simulink model "35-Bus_Network_Electricity_Transmission_Model"  (R2023b)
settings: Solver=VariableStepAuto  StartTime=0.0  StopTime=10  RelTol=1e-3
undefined symbols (not defined in the file): D1, D11, Delta
libraries: spsSeriesRLCBranchLib x47, spsLoadFlowBusLib x35, spsThreePhaseSeriesRLCLoadLib x27, spsDistributedParametersLineLib x22, spsGenericPowerSystemStabilizerLib x20, spsThreePhaseTransformerTwoWindingsLib x19, spsThreePhaseVIMeasurementLib x13, spsSynchronousMachinepuStandardLib x10, spsExcitationSystemLib x10, spsHydraulicTurbineandGovernorLib x10, spsThreePhaseParallelRLCLoadLib x4, spsGroundLib x3
(part 5 of 7)

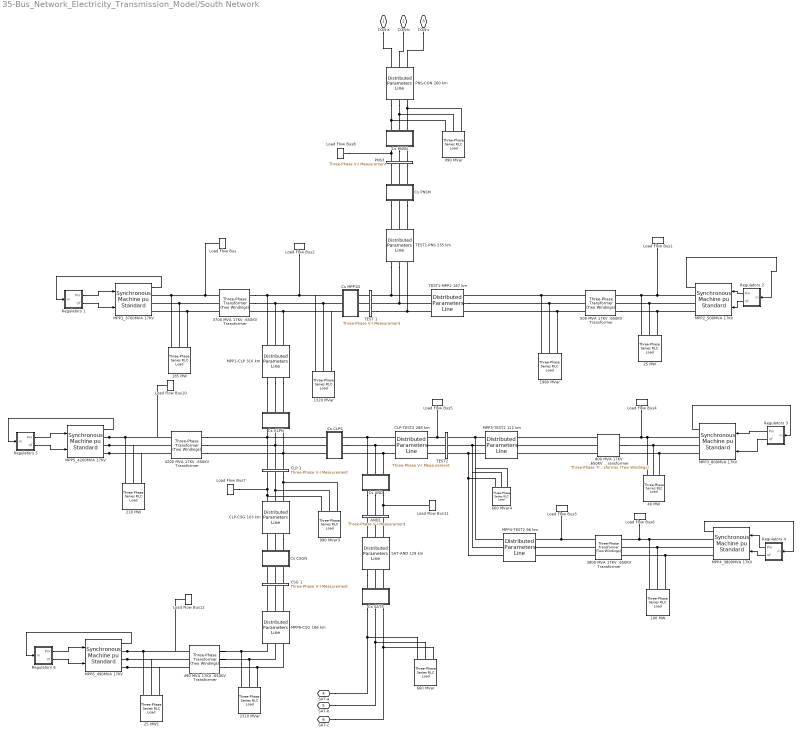
== system 35-Bus_Network_Electricity_Transmission_Model/South Network ==
  " SAT-AND 129 km" : spsDistributedParametersLineLib/Distributed Parameters Line  Phases=3  Length=129  Frequency=60  Resistance=[0.01273 0.3864]/6  Inductance="[0.9337e-3  4.1264e-3]/6"  Capacitance=[12.74e-9 7.751e-9]*6  x1=[-0.00078 -3.83682722016128e-12 0.674511153374435 -1.04249596847644;-0.00072 -3.77067090918174e-12 0.70818806056143 -1.04121442899321;-0.00066 -3.70258545329108e-12 0.741502645650831 -1.03940018496868;-0.0006 -3.63260568626661e-12 0.774437864285324 -1.03705416460361;-0.00054 -3.5607674110502e-12 0.806976866198483 -1.03417756816538;-0.00048 -3.48710738143088e-12 0.839103003835676 -1.03077186737387;-0.00042 -3.41166328324089e-12 0.870799840871265 -1.02683880464853;-0.00036 -3.3344737150749e-12 0.902051160617734 -1.02238039221694;-0.0003 -3.25557816854229e-12 0.932840974322442 -1.01739891108527;-0.00024 -3.17501700806249e-12 0.963153529347768 -1.01189690987132;-0.00018 -3.09283145021379e-12 0.992973317230448 -1.00587720350057;-0.00012 -3.00906354264621e-12 1.022285081616 -0.999342871766043;-6e-05 -2.9237561425691e-12 1.05107382606413 -0.992297257752584]  x2=[-0.00078 2.44939148388225e-11 -0.211095894428946 0.447209046200146;-0.00072 2.42785115163366e-11 -0.22627061958859 0.447871126318045;-0.00066 2.40506868587436e-11 -0.241329580518252 0.448304067292014;-0.0006 2.38105574253482e-11 -0.256265072775263 0.448507647621449;-0.00054 2.35582460708054e-11 -0.271069455085808 0.448481763150892;-0.00048 2.32938818822664e-11 -0.285735153254343 0.448226427123317;-0.00042 2.3017600113335e-11 -0.300254664038695 0.447741770173354;-0.00036 2.27295421148693e-11 -0.314620558988856 0.447028040260454;-0.0003 2.2429855262664e-11 -0.328825488247519 0.446085602542028;-0.00024 2.21186928820502e-11 -0.342862184310398 0.444914939186627;-0.00018 2.17962141694515e-11 -0.35672346574442 0.443516649127255;-0.00012 2.1462584110936e-11 -0.370402240861875 0.441891447754944;-6e-05 2.11179733978064e-11 -0.383891511348658 0.440040166552747]  x3=[-0.00078 4.92364553079132e-13 0.294721852728447 -0.0146104918256409;-0.00072 5.08483648349703e-13 0.292540672457794 -0.0101755439802829;-0.00066 5.24342593990081e-13 0.290209822973581 -0.00573539013860211;-0.0006 5.39933276270636e-13 0.287730496781475 -0.00129230196534861;-0.00054 5.55247718710231e-13 0.285103962350566 0.00315144737346934;-0.00048 5.70278086157137e-13 0.282331563464403 0.00759358437357899;-0.00042 5.85016688797636e-13 0.279414718533485 0.0120318363556098;-0.00036 5.99455986090281e-13 0.276354919869574 0.0164639326278383;-0.0003 6.1358859062377e-13 0.273153732922207 0.0208876056479159;-0.00024 6.27407271896481e-13 0.269812795477775 0.0253005921829855;-0.00018 6.40904960015737e-13 0.26633381682161 0.029700634467593;-0.00012 6.54074749314887e-13 0.262718576863476 0.0340854813588023;-6e-05 6.66909901886376e-13 0.258968925226938 0.0384528894879212]  x4=[-0.00078 -3.24040327625952e-13 -0.286027014427502 0.00132993540133076;-0.00072 -3.4081273578908e-13 -0.283417772465653 -0.00308710233702361;-0.00066 -3.57410777859083e-13 -0.280663528734453 -0.00750256065677927;-0.0006 -3.73825961970941e-13 -0.277765692355886 -0.0119141805278715;-0.00054 -3.90049889813146e-13 -0.27472574591659 -0.016319704884057;-0.00048 -4.06074260924429e-13 -0.271545244709336 -0.0207168797776703;-0.00042 -4.21890876940434e-13 -0.268225815937308 -0.0251034555327854;-0.00036 -4.37491645788148e-13 -0.264769157881604 -0.0294771878961915;-0.0003 -4.52868585825961e-13 -0.261177039032356 -0.033835839185594;-0.00024 -4.68013829927217e-13 -0.257451297183943 -0.0381771794344548;-0.00018 -4.8291962950518e-13 -0.253593838494737 -0.0424989875328837;-0.00012 -4.9757835847736e-13 -0.249606636511881 -0.0467990523639998;-6e-05 -5.11982517167152e-13 -0.245491731161586 -0.0510751739351794]  x5=0.000729548621424508  V1=[2.188e-18 3.182e-07 3.182e-07;377 377 377;0.6306 1.295 -0.2758]  V2=[1.209e-19 1.011e-07 1.011e-07;377 377 377;-2.255 -1.798 2.915]  I1=[1.016e-20 9.164e-09 9.164e-09;377 377 377;2.19 2.786 1.215]  I2=[1.089e-20 9.22e-09 9.22e-09;377 377 377;-0.7019 -0.2685 -1.839]  nHarmo=1  Measurements=None  Decoupling=off  VsMag0=0  VrMag0=0  VsAngle0=0  VrAngle0=0  IsMag0=0  IrMag0=0  IsAngle0=0  IrAngle0=0
      settings: LibrarySourceBlock=sps_lib/Power Grid Elements/Distributed Parameters Line
  1320 MVar : spsThreePhaseSeriesRLCLoadLib/Three-Phase Series RLC Load  LConnTagsString=A|B|C  Configuration=Y (grounded)  NominalVoltage=1000  Vabc=[1e3 1e3 1e3]  Vabcp=[1e3 1e3 1e3]  NominalFrequency=60  UnbalancedPower=off  ActivePower=4400e3  InductivePower=1320e6  CapacitivePower=0  Pabc=[10e3 9e3 11e3]  QLabc=[100 90 110]  QCabc=[100 90 110]  Pabcp=[10e3 9e3 11e3]  QLabcp=[100 90 110]  QCabcp=[100 90 110]  Measurements=None  LoadType=constant Z
  185 MW : spsThreePhaseSeriesRLCLoadLib/Three-Phase Series RLC Load  LConnTagsString=A|B|C  Configuration=Y (grounded)  NominalVoltage=1000  Vabc=[1e3 1e3 1e3]  Vabcp=[1e3 1e3 1e3]  NominalFrequency=60  UnbalancedPower=off  ActivePower=185e6  InductivePower=0  CapacitivePower=0  Pabc=[10e3 9e3 11e3]  QLabc=[100 90 110]  QCabc=[100 90 110]  Pabcp=[10e3 9e3 11e3]  QLabcp=[100 90 110]  QCabcp=[100 90 110]  Measurements=None  LoadType=constant Z
  190 MW : spsThreePhaseSeriesRLCLoadLib/Three-Phase Series RLC Load  LConnTagsString=A|B|C  Configuration=Y (grounded)  NominalVoltage=1000  Vabc=[1e3 1e3 1e3]  Vabcp=[1e3 1e3 1e3]  NominalFrequency=60  UnbalancedPower=off  ActivePower=190e6  InductivePower=0  CapacitivePower=0  Pabc=[10e3 9e3 11e3]  QLabc=[100 90 110]  QCabc=[100 90 110]  Pabcp=[10e3 9e3 11e3]  QLabcp=[100 90 110]  QCabcp=[100 90 110]  Measurements=None  LoadType=constant Z
  1980 MVar : spsThreePhaseSeriesRLCLoadLib/Three-Phase Series RLC Load  LConnTagsString=A|B|C  Configuration=Y (grounded)  NominalVoltage=1000  Vabc=[1e3 1e3 1e3]  Vabcp=[1e3 1e3 1e3]  NominalFrequency=60  UnbalancedPower=off  ActivePower=4400e3  InductivePower=1320e6  CapacitivePower=0  Pabc=[10e3 9e3 11e3]  QLabc=[100 90 110]  QCabc=[100 90 110]  Pabcp=[10e3 9e3 11e3]  QLabcp=[100 90 110]  QCabcp=[100 90 110]  Measurements=None  LoadType=constant Z
  210 MW : spsThreePhaseSeriesRLCLoadLib/Three-Phase Series RLC Load  LConnTagsString=A|B|C  Configuration=Y (grounded)  NominalVoltage=1000  Vabc=[1e3 1e3 1e3]  Vabcp=[1e3 1e3 1e3]  NominalFrequency=60  UnbalancedPower=off  ActivePower=210e6  InductivePower=0  CapacitivePower=0  Pabc=[10e3 9e3 11e3]  QLabc=[100 90 110]  QCabc=[100 90 110]  Pabcp=[10e3 9e3 11e3]  QLabcp=[100 90 110]  QCabcp=[100 90 110]  Measurements=None  LoadType=constant Z
  2310 MVar : spsThreePhaseSeriesRLCLoadLib/Three-Phase Series RLC Load  LConnTagsString=A|B|C  Configuration=Y (grounded)  NominalVoltage=1000  Vabc=[1e3 1e3 1e3]  Vabcp=[1e3 1e3 1e3]  NominalFrequency=60  UnbalancedPower=off  ActivePower=7700e3  InductivePower=2310e6  CapacitivePower=0  Pabc=[10e3 9e3 11e3]  QLabc=[100 90 110]  QCabc=[100 90 110]  Pabcp=[10e3 9e3 11e3]  QLabcp=[100 90 110]  QCabcp=[100 90 110]  Measurements=None  LoadType=constant Z
  25 MW : spsThreePhaseSeriesRLCLoadLib/Three-Phase Series RLC Load  LConnTagsString=A|B|C  Configuration=Y (grounded)  NominalVoltage=1000  Vabc=[1e3 1e3 1e3]  Vabcp=[1e3 1e3 1e3]  NominalFrequency=60  UnbalancedPower=off  ActivePower=25e6  InductivePower=0  CapacitivePower=0  Pabc=[10e3 9e3 11e3]  QLabc=[100 90 110]  QCabc=[100 90 110]  Pabcp=[10e3 9e3 11e3]  QLabcp=[100 90 110]  QCabcp=[100 90 110]  Measurements=None  LoadType=constant Z
  25 MW1 : spsThreePhaseSeriesRLCLoadLib/Three-Phase Series RLC Load  LConnTagsString=A|B|C  Configuration=Y (grounded)  NominalVoltage=1000  Vabc=[1e3 1e3 1e3]  Vabcp=[1e3 1e3 1e3]  NominalFrequency=60  UnbalancedPower=off  ActivePower=25e6  InductivePower=0  CapacitivePower=0  Pabc=[10e3 9e3 11e3]  QLabc=[100 90 110]  QCabc=[100 90 110]  Pabcp=[10e3 9e3 11e3]  QLabcp=[100 90 110]  QCabcp=[100 90 110]  Measurements=None  LoadType=constant Z
  "3700 MVA 17KV :650KV Transformer " : spsThreePhaseTransformerTwoWindingsLib/Three-Phase Transformer (Two Windings)  Winding1Connection=Delta (D1)  Winding2Connection=Yg  CoreType=Three single-phase transformers  SetSaturation=off  Hysteresis=off  DataFile='hysteresis'  SetInitialFlux=off  Measurements=None  UNITS=pu  NominalPower=[ 5500e6 , 60 ]  Winding1=[ 17e3 , 0.002 , 0.08 ]  Winding2=[ 650e3 , 0.002 , 0.08 ]  Rm=500  Lm=500  L0=0.5  Saturation=[ 0,0 ; 0.0024,1.2 ; 1.0,1.52 ]  InitialFluxes=[ 0.8 , -0.8 , 0.7 ]  BreakLoop=off  DiscreteSolver=Trapezoidal iterative  DataType=off  TransfoNumber=1
  3800 MVA 17KV :650KV Transformer : spsThreePhaseTransformerTwoWindingsLib/Three-Phase Transformer (Two Windings)  Winding1Connection=Yg  Winding2Connection=Delta (D1)  CoreType=Three single-phase transformers  SetSaturation=off  Hysteresis=off  DataFile='hysteresis'  SetInitialFlux=off  Measurements=None  UNITS=pu  NominalPower=[ 3800e6 , 60 ]  Winding1=[ 17e3 , 0.002 , 0.08 ]  Winding2=[ 650e3 , 0.002 , 0.08 ]  Rm=500  Lm=500  L0=0.5  Saturation=[ 0,0 ; 0.0024,1.2 ; 1.0,1.52 ]  InitialFluxes=[ 0.8 , -0.8 , 0.7 ]  BreakLoop=off  DiscreteSolver=Trapezoidal iterative  DataType=off  TransfoNumber=1
  40 MW : spsThreePhaseSeriesRLCLoadLib/Three-Phase Series RLC Load  LConnTagsString=A|B|C  Configuration=Y (grounded)  NominalVoltage=1000  Vabc=[1e3 1e3 1e3]  Vabcp=[1e3 1e3 1e3]  NominalFrequency=60  UnbalancedPower=off  ActivePower=40e6  InductivePower=0  CapacitivePower=0  Pabc=[10e3 9e3 11e3]  QLabc=[100 90 110]  QCabc=[100 90 110]  Pabcp=[10e3 9e3 11e3]  QLabcp=[100 90 110]  QCabcp=[100 90 110]  Measurements=None  LoadType=constant Z
  4200 MVA 17KV :650KV Transformer : spsThreePhaseTransformerTwoWindingsLib/Three-Phase Transformer (Two Windings)  Winding1Connection=Delta (D1)  Winding2Connection=Yg  CoreType=Three single-phase transformers  SetSaturation=off  Hysteresis=off  DataFile='hysteresis'  SetInitialFlux=off  Measurements=None  UNITS=pu  NominalPower=[ 4200e6 , 60 ]  Winding1=[ 17e3 , 0.002 , 0.08 ]  Winding2=[ 650e3 , 0.002 , 0.08 ]  Rm=500  Lm=500  L0=0.5  Saturation=[ 0,0 ; 0.0024,1.2 ; 1.0,1.52 ]  InitialFluxes=[ 0.8 , -0.8 , 0.7 ]  BreakLoop=off  DiscreteSolver=Trapezoidal iterative  DataType=off  TransfoNumber=1
  490 MVA 17KV :650KV Transformer : spsThreePhaseTransformerTwoWindingsLib/Three-Phase Transformer (Two Windings)  Winding1Connection=Delta (D1)  Winding2Connection=Yg  CoreType=Three single-phase transformers  SetSaturation=off  Hysteresis=off  DataFile='hysteresis'  SetInitialFlux=off  Measurements=None  UNITS=pu  NominalPower=[ 490e6 , 60 ]  Winding1=[ 17e3 , 0.002 , 0.08 ]  Winding2=[ 650e3 , 0.002 , 0.08 ]  Rm=500  Lm=500  L0=0.5  Saturation=[ 0,0 ; 0.0024,1.2 ; 1.0,1.52 ]  InitialFluxes=[ 0.8 , -0.8 , 0.7 ]  BreakLoop=off  DiscreteSolver=Trapezoidal iterative  DataType=off  TransfoNumber=1
  "500 MVA 17KV :650KV Transformer " : spsThreePhaseTransformerTwoWindingsLib/Three-Phase Transformer (Two Windings)  Winding1Connection=Yg  Winding2Connection=Delta (D1)  CoreType=Three single-phase transformers  SetSaturation=off  Hysteresis=off  DataFile='hysteresis'  SetInitialFlux=off  Measurements=None  UNITS=pu  NominalPower=[ 500e6 , 60 ]  Winding1=[ 17e3 , 0.002 , 0.08 ]  Winding2=[ 650e3 , 0.002 , 0.08 ]  Rm=500  Lm=500  L0=0.5  Saturation=[ 0,0 ; 0.0024,1.2 ; 1.0,1.52 ]  InitialFluxes=[ 0.8 , -0.8 , 0.7 ]  BreakLoop=off  DiscreteSolver=Trapezoidal iterative  DataType=off  TransfoNumber=1
  660 MVar : spsThreePhaseSeriesRLCLoadLib/Three-Phase Series RLC Load  LConnTagsString=A|B|C  Configuration=Y (grounded)  NominalVoltage=1000  Vabc=[1e3 1e3 1e3]  Vabcp=[1e3 1e3 1e3]  NominalFrequency=60  UnbalancedPower=off  ActivePower=2200e3  InductivePower=660e6  CapacitivePower=0  Pabc=[10e3 9e3 11e3]  QLabc=[100 90 110]  QCabc=[100 90 110]  Pabcp=[10e3 9e3 11e3]  QLabcp=[100 90 110]  QCabcp=[100 90 110]  Measurements=None  LoadType=constant Z
  660 MVar4 : spsThreePhaseSeriesRLCLoadLib/Three-Phase Series RLC Load  LConnTagsString=A|B|C  Configuration=Y (grounded)  NominalVoltage=1000  Vabc=[1e3 1e3 1e3]  Vabcp=[1e3 1e3 1e3]  NominalFrequency=60  UnbalancedPower=off  ActivePower=2200e3  InductivePower=660e6  CapacitivePower=0  Pabc=[10e3 9e3 11e3]  QLabc=[100 90 110]  QCabc=[100 90 110]  Pabcp=[10e3 9e3 11e3]  QLabcp=[100 90 110]  QCabcp=[100 90 110]  Measurements=None  LoadType=constant Z
  800 MVA 17KV :650KV Transformer : spsThreePhaseTransformerTwoWindingsLib/Three-Phase Transformer (Two Windings)  Winding1Connection=Yg  Winding2Connection=Yg  CoreType=Three single-phase transformers  SetSaturation=off  Hysteresis=off  DataFile='hysteresis'  SetInitialFlux=off  Measurements=None  UNITS=pu  NominalPower=[ 800e6 , 60 ]  Winding1=[ 17e3 , 0.002 , 0.08 ]  Winding2=[ 650e3 , 0.002 , 0.08 ]  Rm=500  Lm=500  L0=0.5  Saturation=[ 0,0 ; 0.0024,1.2 ; 1.0,1.52 ]  InitialFluxes=[ 0.8 , -0.8 , 0.7 ]  BreakLoop=off  DiscreteSolver=Trapezoidal iterative  DataType=off  TransfoNumber=1
  990 MVar : spsThreePhaseSeriesRLCLoadLib/Three-Phase Series RLC Load  LConnTagsString=A|B|C  Configuration=Y (grounded)  NominalVoltage=1000  Vabc=[1e3 1e3 1e3]  Vabcp=[1e3 1e3 1e3]  NominalFrequency=60  UnbalancedPower=off  ActivePower=2200e3  InductivePower=660e6  CapacitivePower=0  Pabc=[10e3 9e3 11e3]  QLabc=[100 90 110]  QCabc=[100 90 110]  Pabcp=[10e3 9e3 11e3]  QLabcp=[100 90 110]  QCabcp=[100 90 110]  Measurements=None  LoadType=constant Z
  990 MVar3 : spsThreePhaseSeriesRLCLoadLib/Three-Phase Series RLC Load  LConnTagsString=A|B|C  Configuration=Y (grounded)  NominalVoltage=1000  Vabc=[1e3 1e3 1e3]  Vabcp=[1e3 1e3 1e3]  NominalFrequency=60  UnbalancedPower=off  ActivePower=3300e3  InductivePower=990e6  CapacitivePower=0  Pabc=[10e3 9e3 11e3]  QLabc=[100 90 110]  QCabc=[100 90 110]  Pabcp=[10e3 9e3 11e3]  QLabcp=[100 90 110]  QCabcp=[100 90 110]  Measurements=None  LoadType=constant Z
  AND1 : spsThreePhaseVIMeasurementLib/Three-Phase V-I Measurement  VoltageMeasurement=no  SetLabelV=off  LabelV=Vabc  Vpu=off  VpuLL=off  CurrentMeasurement=no  SetLabelI=off  LabelI=Iabc  Ipu=off  Pbase=100e6  Vbase=500e3  OutputType=Complex  PhasorSimulation=off  PSBequivalent=0
  CLP 1 : spsThreePhaseVIMeasurementLib/Three-Phase V-I Measurement  VoltageMeasurement=no  SetLabelV=off  LabelV=Vabc  Vpu=off  VpuLL=off  CurrentMeasurement=no  SetLabelI=off  LabelI=Iabc  Ipu=off  Pbase=100e6  Vbase=500e3  OutputType=Complex  PhasorSimulation=off  PSBequivalent=0
  CLP-CSG 103 km : spsDistributedParametersLineLib/Distributed Parameters Line  Phases=3  Length=103  Frequency=60  Resistance=[0.01273 0.3864]/6  Inductance="[0.9337e-3  4.1264e-3]/6"  Capacitance=[12.74e-9 7.751e-9]*6  x1=[-0.0006 -2.86875553089972e-12 0.579434084847249 -0.777616675486006;-0.00054 -2.78336212016804e-12 0.603536759120955 -0.77512217164524;-0.00048 -2.69654468994506e-12 0.627330652836618 -0.772231100978851;-0.00042 -2.60834765763229e-12 0.650803592598553 -0.76894494261201;-0.00036 -2.51881614646115e-12 0.673943569217046 -0.76526537780406;-0.0003 -2.42799596240711e-12 0.696738743852482 -0.761194289088347;-0.00024 -2.3359335707545e-12 0.719177454072312 -0.756733759309083;-0.00018 -2.242676072324e-12 0.741248219817767 -0.751886070555725;-0.00012 -2.14827117937501e-12 0.762939749277271 -0.746653702995413;-6e-05 -2.05276719119516e-12 0.784240944663539 -0.741039333604074]  x2=[-0.0006 -2.50536213326479e-12 1.13677413168681 -1.46477585686009;-0.00054 -2.38568590540881e-12 1.18226888987211 -1.46001833109431;-0.00048 -2.26478911656121e-12 1.22715877744753 -1.45451383297231;-0.00042 -2.14273361975309e-12 1.27142082791713 -1.44826517869704;-0.00036 -2.01958186083194e-12 1.31503239599801 -1.44127556519548;-0.0003 -1.89539684651321e-12 1.35797116920609 -1.43354856848305;-0.00024 -1.77024211214489e-12 1.40021517927158 -1.42508814183406;-0.00018 -1.64418168920169e-12 1.44174281337835 -1.41589861375911;-0.00012 -1.51728007252531e-12 1.48253282522146 -1.40598468579055;-6e-05 -1.38960218732771e-12 1.52256434587713 -1.39535143007714]  x3=[-0.0006 -7.54690409347094e-14 -0.142926241061313 -0.0366777002010042;-0.00054 -7.42619788377903e-14 -0.140121811441698 -0.0392014264931644;-0.00048 -7.30169229402942e-14 -0.137245692914197 -0.0417050966111716;-0.00042 -7.17345102358242e-14 -0.134299356954192 -0.044187429631131;-0.00036 -7.04153968304162e-14 -0.131284310961602 -0.0466471555456012;-0.0003 -6.90602576068629e-14 -0.128202097489669 -0.049083015913354;-0.00024 -6.7669785879431e-14 -0.125054293455758 -0.0514937645032156;-0.00018 -6.62446930391493e-14 -0.121842509334578 -0.0538781679316621;-0.00012 -6.47857081898477e-14 -0.118568388334231 -0.0562350062938406;-6e-05 -6.32935777751338e-14 -0.11523360555552 -0.0585630737876958]  x4=[-0.0006 2.5096768503781e-14 0.176233491587121 -0.0132782448226382;-0.00054 2.54022915681483e-14 0.175024690970161 -0.0106694613096422;-0.00048 2.5694818350769e-14 0.173726344487216 -0.00805521910309131;-0.00042 2.59741991895358e-14 0.172339116396338 -0.00543685569760391;-0.00036 2.62402911480492e-14 0.17086371642905 -0.00281571069628007;-0.0003 2.64929580887464e-14 0.169300899427239 -0.000193125125335665;-0.00024 2.67320707425518e-14 0.16765146495696 0.0024295592519914;-0.00018 2.69575067750134e-14 0.165916256899366 0.00505100062191206;-0.00012 2.71691508488915e-14 0.164096163018962 0.00766985780658279;-6e-05 2.73668946831672e-14 0.16219211450941 0.010284790950277]  x5=0.000582507814005615  V1=[1.056e-22 6.221e-12 6.221e-12;377 377 377;0.3647 1.373 -0.1974]  V2=[1.588e-22 9.824e-12 9.824e-12;377 377 377;0.3755 1.375 -0.1957]  I1=[3.913e-25 1.044e-13 1.044e-13;377 377 377;-0.5956 0.0636 -1.507]  I2=[3.097e-25 1.021e-13 1.021e-13;377 377 377;1.525 2.624 1.053]  nHarmo=1  Measurements=None  Decoupling=off  VsMag0=0  VrMag0=0  VsAngle0=0  VrAngle0=0  IsMag0=0  IrMag0=0  IsAngle0=0  IrAngle0=0
      settings: LibrarySourceBlock=sps_lib/Power Grid Elements/Distributed Parameters Line
  CLP-TEST2 288 km : spsDistributedParametersLineLib/Distributed Parameters Line  Phases=3  Length=288  Frequency=60  Resistance=[0.01273 0.3864]/6  Inductance="[0.9337e-3  4.1264e-3]/6"  Capacitance=[12.74e-9 7.751e-9]*6  x1=[-0.00168 -1.46851592292869e-14 0 0;-0.00162 -1.46801716193227e-14 0 0;-0.00156 -1.46676733622997e-14 0 0;-0.0015 -1.4647670852557e-14 0 0;-0.00144 -1.46201743237484e-14 0 0;-0.00138 -1.45851978436059e-14 0 0;-0.00132 -1.45427593067432e-14 0 0;-0.00126 -1.44928804254999e-14 0 0;-0.0012 -1.44355867188333e-14 0 0;-0.00114 -1.43709074992623e-14 0 0;-0.00108 -1.42988758578708e-14 0 0;-0.00102 -1.42195286473777e-14 -0.00333231369299481 -0.0123382133221417;-0.00096 -1.41329064632818e-14 -0.00304195535243525 -0.0124269013961661;-0.0009 -1.40390536230933e-14 -0.00275004069130851 -0.0125092316378136;-0.00084 -1.39380181436592e-14 -0.00245671905854919 -0.0125851619254111;-0.00078 -1.3829851716598e-14 -0.00216214052292456 -0.0126546534116205;-0.00072 -1.37146096818522e-14 -0.00186645579625664 -0.0127176705433135;-0.00066 -1.35923509993764e-14 -0.00156981615631522 -0.0127741810797609;-0.0006 -1.34631382189715e-14 -0.00127237336942136 -0.0128241561091282;-0.00054 -1.33270374482836e-14 -0.00097427961280095 -0.0128675700632669;-0.00048 -1.31841183189818e-14 -0.000675687396728012 -0.0129044007307959;-0.00042 -1.30344539511335e-14 -0.00037674948649764 -0.0129346292684651;-0.00036 -1.28781209157948e-14 -7.76188242684462e-05 -0.0129582402107961;-0.0003 -1.27151991958353e-14 0.000221551549185474 -0.0129752214779945;-0.00024 -1.25457721450173e-14 0.00052060857277303 -0.0129855643821302;-0.00018 -1.23699264453507e-14 0.000819399243395014 -0.0129892636315824;-0.00012 -1.21877520627447e-14 0.00111777069422332 -0.0129863173337467;-6e-05 -1.19993422009796e-14 0.00141557027291043 -0.0129767269960034]  x2=[-0.00168 1.19189119305779e-11 0 0;-0.00162 1.20216070434036e-11 0 0;-0.00156 1.21181516799321e-11 0 0;-0.0015 1.22084964461435e-11 0 0;-0.00144 1.2292595119986e-11 0 0;-0.00138 1.2370404675024e-11 0 0;-0.00132 1.24418853024515e-11 0 0;-0.00126 1.25070004314587e-11 0 0;-0.0012 1.25657167479423e-11 0 0;-0.00114 1.26180042115499e-11 0 0;-0.00108 1.2663836071049e-11 0 0;-0.00102 1.27031888780134e-11 0.391127559553685 -0.606252923162327;-0.00096 1.27360424988198e-11 0.410722433320571 -0.605525073329179;-0.0009 1.27623801249488e-11 0.430107173901292 -0.604487425679699;-0.00084 1.27821882815842e-11 0.449271863704378 -0.603140511093598;-0.00078 1.27954568345071e-11 0.468206697720403 -0.601485018677266;-0.00072 1.28021789952806e-11 0.48690198853841 -0.599521795411214;-0.00066 1.2802351324723e-11 0.505348171302166 -0.59725184571674;-0.0006 1.27959737346675e-11 0.523535808603723 -0.594676330942052;-0.00054 1.27830494880069e-11 0.541455595311769 -0.591796568768099;-0.00048 1.27635851970246e-11 0.559098363332305 -0.588614032534421;-0.00042 1.27375908200116e-11 0.57645508629921 -0.585130350485362;-0.00036 1.27050796561714e-11 0.593516884192299 -0.581347304937029;-0.0003 1.26660683388163e-11 0.610275027880504 -0.577266831365427;-0.00024 1.2620576826857e-11 0.626720943587859 -0.572891017416233;-0.00018 1.25686283945917e-11 0.642846217280003 -0.568222101836721;-0.00012 1.25102496197981e-11 0.658642598968955 -0.563262473330371;-6e-05 1.24454703701362e-11 0.674102006933958 -0.558014669334772]  x3=[-0.00168 -2.46538549187003e-14 0 0;-0.00162 -2.09683351939942e-14 0 0;-0.00156 -1.72720876815525e-14 0 0;-0.0015 -1.35670034499015e-14 0 0;-0.00144 -9.85497808859615e-15 0 0;-0.00138 -6.13791073840156e-15 0 0;-0.00132 -2.41770311965766e-15 0 0;-0.00126 1.30374144067627e-15 0 0;-0.0012 5.02451898279877e-15 0 0;-0.00114 8.74272588816724e-15 0 0;-0.00108 1.24564598534243e-14 0 0;-0.00102 1.61638208636515e-14 -0.0508652629432111 -0.00327294157959855;-0.00096 1.98629121644517e-14 -0.0502690146140841 -0.00408129610717447;-0.0009 2.35518412323642e-14 -0.049647047728216 -0.00488756256824828;-0.00084 2.72287207431143e-14 -0.0489996804953581 -0.00569132846200041;-0.00078 3.08916695372032e-14 -0.0483272441205488 -0.00649218256694771;-0.00072 3.45388135823445e-14 -0.0476300826346627 -0.00728971515133202;-0.00066 3.81682869322531e-14 -0.0469085527183979 -0.00808351818274646;-0.0006 4.17782326812984e-14 -0.046163023519792 -0.00887318553689237;-0.00054 4.53668039145309e-14 -0.0453938764653588 -0.00965831320535999;-0.00048 4.89321646525987e-14 -0.0446015050649435 -0.0104384995023266;-0.00042 5.24724907910676e-14 -0.0437863147103959 -0.0112133452700666;-0.00036 5.59859710336678e-14 -0.0429487224681645 -0.0119824540831676;-0.0003 5.94708078189853e-14 -0.0420891568659171 -0.0127454324513493;-0.00024 6.29252182401284e-14 -0.041208057673299 -0.0135018900207805;-0.00018 6.63474349568955e-14 -0.0403058756769378 -0.0142514397737907;-0.00012 6.97357070999791e-14 -0.0393830724498134 -0.0149936982268764;-6e-05 7.30883011667426e-14 -0.0384401201151081 -0.0157282856268975]  x4=[-0.00168 1.00387184624451e-13 0 0;-0.00162 9.81055530042471e-14 0 0;-0.00156 9.57737287703444e-14 0 0;-0.0015 9.33929049271079e-14 0 0;-0.00144 9.09642995480081e-14 0 0;-0.00138 8.84891551524326e-14 0 0;-0.00132 8.59687380699895e-14 0 0;-0.00126 8.34043377926301e-14 0 0;-0.0012 8.07972663149211e-14 0 0;-0.00114 7.81488574628035e-14 0 0;-0.00108 7.54604662111832e-14 0 0;-0.00102 7.27334679907001e-14 0.055687205911254 -0.01038556626525;-0.00096 6.99692579840329e-14 0.0555646955243274 -0.00962151775077783;-0.0009 6.71692504120979e-14 0.0554137572124531 -0.00885254669003919;-0.00084 6.43348778105071e-14 0.0552344681984603 -0.00807904650283767;-0.00078 6.14675902966565e-14 0.0550269202099215 -0.00730141292616168;-0.00072 5.85688548278197e-14 0.0547912194322228 -0.00652004381171807;-0.00066 5.56401544506249e-14 0.0545274864542373 -0.00573533892238383;-0.0006 5.26829875423014e-14 0.0542358562066296 -0.00494769972768002;-0.00054 4.96988670440815e-14 0.0539164778928233 -0.00415752919837254;-0.00048 4.66893196871524e-14 0.053569514912665 -0.00336523160030487;-0.00042 4.3655885211552e-14 0.0531951447788265 -0.00257121228756816;-0.00036 4.06001155784093e-14 0.052793559025986 -0.00177587749511459;-0.0003 3.75235741759328e-14 0.0523649631128349 -0.000979634130920067;-0.00024 3.44278350195519e-14 0.0519095763169621 -0.000182889567802613;-0.00018 3.13144819466219e-14 0.0514276316226668 0.00061394856499714;-0.00012 2.81851078061028e-14 0.05091937560176 0.00141047259036658;-6e-05 2.50413136436292e-14 0.0503850682874134 0.00220627499189624]  x5=0.00162875971294774  V1=[1.245e-23 7.93e-13 7.93e-13;377 377 377;-1.837 -1.972 2.74]  V2=[6.065e-20 5.187e-08 5.187e-08;377 377 377;-2.594 -2.004 2.709]  I1=[1.297e-22 5.199e-10 5.199e-10;377 377 377;2.342 2.744 1.173]  I2=[1.117e-22 5.13e-10 5.13e-10;377 377 377;-1.44 -0.7735 -2.344]  nHarmo=1  Measurements=None  Decoupling=off  VsMag0=0  VrMag0=0  VsAngle0=0  VrAngle0=0  IsMag0=0  IrMag0=0  IsAngle0=0  IrAngle0=0
      settings: LibrarySourceBlock=sps_lib/Power Grid Elements/Distributed Parameters Line
  CSG 1 : spsThreePhaseVIMeasurementLib/Three-Phase V-I Measurement  VoltageMeasurement=no  SetLabelV=off  LabelV=Vabc  Vpu=off  VpuLL=off  CurrentMeasurement=no  SetLabelI=off  LabelI=Iabc  Ipu=off  Pbase=100e6  Vbase=500e3  OutputType=Complex  PhasorSimulation=off  PSBequivalent=0
  Cs AND : Subsystem
  Cs CLPN : Subsystem
  Cs CLPS : Subsystem
  Cs CSGN : Subsystem
  Cs MPP1D : Subsystem
  Cs PNSM : Subsystem
  Cs PNSN : Subsystem
  Cs SATS : Subsystem
  Load Flow Bus : spsLoadFlowBusLib/Load Flow Bus  LConnTagsString=a  Phases=single  Connectors=on one side  ID=BUS_1  Vbase=17e3  Vref=1  Vangle=0  VLF=1  VLFb=1  VLFc=1  angleLF=0  angleLFb=0  angleLFc=0
  Load Flow Bus1 : spsLoadFlowBusLib/Load Flow Bus  LConnTagsString=a  Phases=single  Connectors=on one side  ID=BUS_2  Vbase=17e3  Vref=1  Vangle=0  VLF=1  VLFb=1  VLFc=1  angleLF=0  angleLFb=0  angleLFc=0
  Load Flow Bus10 : spsLoadFlowBusLib/Load Flow Bus  LConnTagsString=a  Phases=single  Connectors=on one side  ID=BUS_5  Vbase=17e3  Vref=1  Vangle=0  VLF=1  VLFb=1  VLFc=1  angleLF=0  angleLFb=0  angleLFc=0
  Load Flow Bus11 : spsLoadFlowBusLib/Load Flow Bus  LConnTagsString=a  Phases=single  Connectors=on one side  ID=BUS_11  Vbase=650e3  Vref=1.031  Vangle=17.31  VLF=1  VLFb=1  VLFc=1  angleLF=0  angleLFb=0  angleLFc=0
  Load Flow Bus12 : spsLoadFlowBusLib/Load Flow Bus  LConnTagsString=a  Phases=single  Connectors=on one side  ID=BUS_6  Vbase=17e3  Vref=1  Vangle=0  VLF=1  VLFb=1  VLFc=1  angleLF=0  angleLFb=0  angleLFc=0
  Load Flow Bus2 : spsLoadFlowBusLib/Load Flow Bus  LConnTagsString=a  Phases=single  Connectors=on one side  ID=BUS_7  Vbase=650e3  Vref=1  Vangle=0  VLF=1  VLFb=1  VLFc=1  angleLF=0  angleLFb=0  angleLFc=0
  Load Flow Bus3 : spsLoadFlowBusLib/Load Flow Bus  LConnTagsString=a  Phases=single  Connectors=on one side  ID=BUS_9  Vbase=650e3  Vref=1.031  Vangle=17.31  VLF=1  VLFb=1  VLFc=1  angleLF=0  angleLFb=0  angleLFc=0
  Load Flow Bus4 : spsLoadFlowBusLib/Load Flow Bus  LConnTagsString=a  Phases=single  Connectors=on one side  ID=BUS_3  Vbase=17e3  Vref=1  Vangle=0  VLF=1  VLFb=1  VLFc=1  angleLF=0  angleLFb=0  angleLFc=0
  Load Flow Bus5 : spsLoadFlowBusLib/Load Flow Bus  LConnTagsString=a  Phases=single  Connectors=on one side  ID=BUS_8  Vbase=650e3  Vref=1.031  Vangle=17.31  VLF=1  VLFb=1  VLFc=1  angleLF=0  angleLFb=0  angleLFc=0
  Load Flow Bus6 : spsLoadFlowBusLib/Load Flow Bus  LConnTagsString=a  Phases=single  Connectors=on one side  ID=BUS_4  Vbase=17e3  Vref=1  Vangle=0  VLF=1  VLFb=1  VLFc=1  angleLF=0  angleLFb=0  angleLFc=0
  Load Flow Bus7 : spsLoadFlowBusLib/Load Flow Bus  LConnTagsString=a  Phases=single  Connectors=on one side  ID=BUS_10  Vbase=650e3  Vref=1.031  Vangle=17.31  VLF=1  VLFb=1  VLFc=1  angleLF=0  angleLFb=0  angleLFc=0
  Load Flow Bus8 : spsLoadFlowBusLib/Load Flow Bus  LConnTagsString=a  Phases=single  Connectors=on one side  ID=BUS_12  Vbase=650e3  Vref=1  Vangle=0  VLF=1  VLFb=1  VLFc=1  angleLF=0  angleLFb=0  angleLFc=0
  MPP1-CLP 310 km : spsDistributedParametersLineLib/Distributed Parameters Line  Phases=3  Length=310  Frequency=60  Resistance=[0.01273 0.3864]/6  Inductance="[0.9337e-3  4.1264e-3]/6"  Capacitance=[12.74e-9 7.751e-9]*6  x1=[-0.0018 7.96598431649033e-13 0.453171737691257 -2.03578508071873;-0.00174 8.42533660402322e-13 0.499101481478359 -2.02501547391971;-0.00168 8.88037833366716e-13 0.544775875725202 -2.01320983178625;-0.00162 9.33087669766509e-13 0.590171552567722 -2.00037419430301;-0.00156 9.7766012127297e-13 0.635265286738833 -1.9865151284193;-0.0015 1.02173238379631e-12 0.680034007450895 -1.97163972468931;-0.00144 1.06528190915265e-12 0.724454810199162 -1.95575559364445;-0.00138 1.10828641660012e-12 0.768504968480145 -1.93887086189968;-0.00132 1.15072390423809e-12 0.812161945418915 -1.92099416799574;-0.00126 1.19257266026371e-12 0.85540340529938 -1.90213465797957;-0.0012 1.23381127408013e-12 0.898207224991658 -1.88230198072497;-0.00114 1.27441864725052e-12 0.940551505270668 -1.86150628299609;-0.00108 1.31437400429243e-12 0.982414582020188 -1.83975820425615;-0.00102 1.3536569033069e-12 1.02377503731661 -1.81706887122408;-0.00096 1.39224724643694e-12 1.06461171038676 -1.79344989218193;-0.0009 1.43012529014993e-12 1.10490370843411 -1.76891335103579;-0.00084 1.4672716553388e-12 1.14463041732795 -1.7434718011335;-0.00078 1.50366733723674e-12 1.18377151214995 -1.71713825884209;-0.00072 1.53929371514037e-12 1.22230696759274 -1.6899261968884;-0.00066 1.57413256193645e-12 1.26021706820529 -1.66184953746613;-0.0006 1.60816605342723e-12 1.2974824184796 -1.63292264511305;-0.00054 1.64137677744957e-12 1.3340839527739 -1.60316031936178;-0.00048 1.67374774278342e-12 1.37000294506693 -1.57257778716813;-0.00042 1.70526238784476e-12 1.40522101853852 -1.54119069512067;-0.00036 1.73590458915886e-12 1.43972015497152 -1.50901510143566;-0.0003 1.7656586696093e-12 1.47348270397027 -1.47606746774136;-0.00024 1.79450940645876e-12 1.50649139199084 -1.44236465065597;-0.00018 1.82244203913715e-12 1.5387293311785 -1.40792389316347;-0.00012 1.84944227679346e-12 1.57018002800789 -1.37276281579179;-6e-05 1.8754963056072e-12 1.60082739172135 -1.3368994075978]  x2=[-0.0018 3.2722449946723e-12 0.00643015913645979 -1.11050535754396;-0.00174 3.39133271800325e-12 0.0598956088857668 -1.12936416224046;-0.00168 3.50868537285104e-12 0.113330414934825 -1.1476451633633;-0.00162 3.62424291942903e-12 0.166707239049496 -1.16533900801453;-0.00156 3.73794623636112e-12 0.219998772660274 -1.18243664369626;-0.0015 3.84973715092939e-12 0.273177750833849 -1.19892932294216;-0.00144 3.95955846883629e-12 0.326216966222353 -1.21480860779278;-0.00138 4.06735400346629e-12 0.379089282983142 -1.23006637411257;-0.00132 4.17306860463207e-12 0.431767650661991 -1.24469481574635;-0.00126 4.27664818679027e-12 0.484225118032613 -1.25868644851308;-0.0012 4.37803975671273e-12 0.536434846885398 -1.27203411403489;-0.00114 4.47719144059879e-12 0.58837012575834 -1.28473098339948;-0.00108 4.57405251061486e-12 0.640004383603115 -1.29677056065387;-0.00102 4.66857341084771e-12 0.691311203379317 -1.30814668612785;-0.00096 4.76070578265827e-12 0.742264335569907 -1.31885353958545;-0.0009 4.85040248942268e-12 0.792837711610952 -1.32888564320257;-0.00084 4.93761764064837e-12 0.84300545722878 -1.33823786436966;-0.00078 5.02230661545243e-12 0.892741905677741 -1.34690541831754;-0.00072 5.10442608539046e-12 0.942021610871782 -1.35488387056546;-0.00066 5.18393403662426e-12 0.990819360403144 -1.36216913918982;-0.0006 5.26078979141683e-12 1.03911018844149 -1.36875749691258;-0.00054 5.3349540289439e-12 1.08686938850687 -1.37464557300818;-0.00048 5.40638880541114e-12 1.13407252611006 -1.37983035502811;-0.00042 5.47505757346695e-12 1.18069545125365 -1.38430919034207;-0.00036 5.54092520090075e-12 1.22671431078762 -1.38807978749517;-0.0003 5.60395798861724e-12 1.27210556061313 -1.39114021738021;-0.00024 5.66412368787751e-12 1.31684597772801 -1.39348891422472;-0.00018 5.72139151679809e-12 1.36091267210817 -1.39512467639201;-0.00012 5.77573217609953e-12 1.40428309841851 -1.39604666699591;-6e-05 5.82711786409641e-12 1.44693506754753 -1.396254414329]  x3=[-0.0018 -3.11804643397621e-14 -0.0184752210268118 0.0279530842164615;-0.00174 -2.99439906288817e-14 -0.0179666859209005 0.029078498416484;-0.00168 -2.86921970190943e-14 -0.0174489587264859 0.0301890355194078;-0.00162 -2.7425723951141e-14 -0.0169223043223671 0.0312841273539306;-0.00156 -2.61452193760453e-14 -0.0163869921546688 0.032363213650835;-0.0015 -2.48513384236086e-14 -0.0158432960989873 0.0334257423296321;-0.00144 -2.35447430672345e-14 -0.0152914943202711 0.0344711697810167;-0.00138 -2.22261017852504e-14 -0.0147318691305064 0.0354989611449873;-0.00132 -2.08960892189018e-14 -0.0141647068442809 0.0365085905844908;-0.00126 -1.95553858271934e-14 -0.0135902976323001 0.03749954155445;-0.0012 -1.82046775387539e-14 -0.0130089353729308 0.0384713070660382;-0.00114 -1.68446554009018e-14 -0.0124209175018472 0.0394233899460633;-0.00108 -1.54760152260932e-14 -0.0118265448598576 0.0403553030913316;-0.00102 -1.4099457235931e-14 -0.0112261215389882 0.041266569717858;-0.00096 -1.27156857029189e-14 -0.0106199547269045 0.0421567236047983;-0.0009 -1.13254085901423e-14 -0.0100083545497484 0.0430253093329756;-0.00084 -9.92933718906149e-15 -0.00939163391347153 0.0438718825178819;-0.00078 -8.52818575560172e-15 -0.00877010834374707 0.0446960100370329;-0.00072 -7.12267114472663e-15 -0.00814409582454097 0.0454972702515616;-0.00066 -5.71351244368207e-15 -0.00751391663542545 0.0462752532219367;-0.0006 -4.30143060409774e-15 -0.00687989318771804 0.0470295609176952;-0.00054 -2.88714807313506e-15 -0.00624234985952997 0.0477598074210817;-0.00048 -1.4713884238698e-15 -0.00560161282980841 0.0484656191244919;-0.00042 -5.48759850987584e-17 -0.00495800991145721 0.0491466349216162;-0.00036 1.36166452924025e-15 -0.00431187038362182 0.0498025063921893;-0.0003 2.77750839084544e-15 -0.00366352482322397 0.0504328979802477;-0.00024 4.19193122783541e-15 -0.0030133049358324 0.0510374871658065;-0.00018 5.60420939535124e-15 -0.00236154338595619 0.051615964629867;-0.00012 7.01362034578652e-15 -0.00170857362684741 0.0521680344126694;-6e-05 8.4194429984561e-15 -0.00105472972990033 0.052693414065112]  x4=[-0.0018 4.15748811858138e-14 0.00877100112689456 -0.0951489313324;-0.00174 4.17762594653909e-14 0.0104928973321642 -0.0967719930667223;-0.00168 4.1956264238689e-14 0.0122094251772722 -0.0983455444612507;-0.00162 4.21148034119401e-14 0.0139197064548553 -0.0998687804580161;-0.00156 4.22517958735734e-14 0.0156228661534095 -0.101340921741336;-0.0015 4.23671715357144e-14 0.0173180329049623 -0.102761215136529;-0.00144 4.24608713700424e-14 0.0190043394308804 -0.104128933995248;-0.00138 4.25328474379909e-14 0.0206809229855858 -0.105443378567254;-0.00132 4.25830629152734e-14 0.0223469257979524 -0.106703876358416;-0.00126 4.26114921107238e-14 0.0240014955101569 -0.107909782474772;-0.0012 4.26181204794407e-14 0.0256437856137618 -0.10906047995247;-0.00114 4.26029446302279e-14 0.0272729558828041 -0.110155380073418;-0.00108 4.25659723273303e-14 0.0288881728036704 -0.111193922666483;-0.00102 4.25072224864614e-14 0.0304886100015383 -0.112175576394085;-0.00096 4.24267251651252e-14 0.0320734486631647 -0.113099839024037;-0.0009 4.23245215472389e-14 0.0336418779558058 -0.1139662376865;-0.00084 4.22006639220617e-14 0.0351930954420543 -0.114774329115908;-0.00078 4.20552156574433e-14 0.036726307490381 -0.115523699877755;-0.00072 4.18882511674036e-14 0.0382407296811715 -0.116213966580112;-0.00066 4.16998558740608e-14 0.0397355872080496 -0.11684477606978;-0.0006 4.1490126163928e-14 0.0412101152742829 -0.117415805612967;-0.00054 4.12591693386004e-14 0.0426635594840665 -0.117926763060407;-0.00048 4.10071035598574e-14 0.0440951762284861 -0.11837738699683;-0.00042 4.0734057789209e-14 0.045504233065962 -0.118767446874703;-0.00036 4.04401717219167e-14 0.0468900090969799 -0.119096743132184;-0.0003 4.01255957155231e-14 0.0482517953329159 -0.119365107295225;-0.00024 3.97904907129257e-14 0.049588895058769 -0.119572402063759;-0.00018 3.94350281600358e-14 0.0509006241896126 -0.119718521381954;-0.00012 3.90593899180637e-14 0.0521863116205854 -0.119803390492466;-6e-05 3.8663768170475e-14 0.0534452995702409 -0.119826965974689]  x5=0.0017531788576868  V1=[1.492e-21 4.488e-11 4.488e-11;377 377 377;2.889 -1.992 2.721]  V2=[1.003e-22 1.265e-11 1.265e-11;377 377 377;0.8549 1.122 -0.4483]  I1=[2.499e-24 5.251e-13 5.251e-13;377 377 377;-2.215 -0.7076 -2.278]  I2=[3.136e-24 5.274e-13 5.274e-13;377 377 377;1.561 2.663 1.092]  nHarmo=1  Measurements=None  Decoupling=off  VsMag0=0  VrMag0=0  VsAngle0=0  VrAngle0=0  IsMag0=0  IrMag0=0  IsAngle0=0  IrAngle0=0
      settings: LibrarySourceBlock=sps_lib/Power Grid Elements/Distributed Parameters Line
  MPP1_3700MVA 17KV : spsSynchronousMachinepuStandardLib/Synchronous Machine pu Standard  PresetModel=No  MechanicalLoad=Mechanical power Pm  ShowDetailedParameters=on  RotorType=Salient-pole  Units=per unit standard parameters  MeasurementBus=off  NominalParameters=[3700e6 17000 60]  Reactances1=[ 1.81, 0.3, 0.23, 1.76, 0.65, 0.25, 0.15 ]  Reactances2=[2.24 0.17 0.12 1.02 0.13 0.08]  dAxisTimeConstants=Short-circuit  qAxisTimeConstants=Open-circuit  TimeConstants1="[ 4.4849  0.0681  0.1  ]"  TimeConstants2=[ 8.0, 0.03, 1.0, 0.07 ]  TimeConstants3="[  4.49  0.0681  0.0513  ]"  TimeConstants4=[ 8.0, 0.03, 0.3371, 0.0295 ]  TimeConstants5=[ 1.01, 0.053, 0.1 ]  TimeConstants6=[ 1.3201, 0.023, 1.0, 0.07 ]  TimeConstants7=[0.012 0.003 0.003]  TimeConstants8=[ 1.3201, 0.0231, 0.3371, 0.0295 ]  StatorResistance=0.037875  Mechanical=[3.8 0 28]  PolePairs=20  InitialConditions="[  0 -113.876 0.604539 0.604539 0.604539 -42.1129 -162.113 77.8871 1.28555]"  SetSaturation=off  Saturation=[0.6404,0.7127,0.8441,0.9214,0.9956,1.082,1.19,1.316,1.457;0.7,0.7698,0.8872,0.9466,0.9969,1.046,1.1,1.151,1.201]  LoadFlowParameters=[1,0,0,0,0]  TsPowergui=0  TsBlock=-1  IterativeModel=Trapezoidal non iterative  IterativeDiscreteModel=Trapezoidal non iterative  BusType=PV  Pref=3000e6  Qref=0  Qmin=-inf  Qmax=inf  PLF=0  QLF=0
  MPP2_500MVA 17KV : spsSynchronousMachinepuStandardLib/Synchronous Machine pu Standard  PresetModel=No  MechanicalLoad=Mechanical power Pm  ShowDetailedParameters=on  RotorType=Salient-pole  Units=per unit standard parameters  MeasurementBus=off  NominalParameters=[500e6 17000 60]  Reactances1=[ 1.81, 0.3, 0.23, 1.76, 0.65, 0.25, 0.15 ]  Reactances2=[2.24 0.17 0.12 1.02 0.13 0.08]  dAxisTimeConstants=Short-circuit  qAxisTimeConstants=Open-circuit  TimeConstants1="[ 4.4849  0.0681  0.1  ]"  TimeConstants2=[ 8.0, 0.03, 1.0, 0.07 ]  TimeConstants3="[  4.49  0.0681  0.0513  ]"  TimeConstants4=[ 8.0, 0.03, 0.3371, 0.0295 ]  TimeConstants5=[ 1.01, 0.053, 0.1 ]  TimeConstants6=[ 1.3201, 0.023, 1.0, 0.07 ]  TimeConstants7=[0.012 0.003 0.003]  TimeConstants8=[ 1.3201, 0.0231, 0.3371, 0.0295 ]  StatorResistance=0.037875  Mechanical=[3.8 0 28]  PolePairs=20  InitialConditions=[ 0 -107.876 0.604539 0.604539 0.604539 -42.1129 -162.113 77.8871 1.28555]  SetSaturation=off  Saturation=[0.6404,0.7127,0.8441,0.9214,0.9956,1.082,1.19,1.316,1.457;0.7,0.7698,0.8872,0.9466,0.9969,1.046,1.1,1.151,1.201]  LoadFlowParameters=[1,0,0,0,0]  TsPowergui=0  TsBlock=-1  IterativeModel=Trapezoidal non iterative  IterativeDiscreteModel=Trapezoidal non iterative  BusType=PV  Pref=4100e6  Qref=0  Qmin=-inf  Qmax=inf  PLF=0  QLF=0
  MPP3-TEST2 111 km : spsDistributedParametersLineLib/Distributed Parameters Line  Phases=3  Length=111  Frequency=60  Resistance=[0.01273 0.3864]/6  Inductance="[0.9337e-3  4.1264e-3]/6"  Capacitance=[12.74e-9 7.751e-9]*6  x1=[-0.00066 -2.03193286930705e-13 0 0;-0.0006 -1.99002956379909e-13 0 0;-0.00054 -1.94710812239478e-13 0 0;-0.00048 -1.90319050449662e-13 0 0;-0.00042 -1.85829917916945e-13 -8.60278619544915 -23.3411482282694;-0.00036 -1.8124571136448e-13 -8.04386477267868 -23.6040048194719;-0.0003 -1.76568776157045e-13 -7.48082796005699 -23.8547851656568;-0.00024 -1.71801505101112e-13 -6.91396381762111 -24.0933609629652;-0.00018 -1.66946337220642e-13 -6.34356236354079 -24.3196101516109;-0.00012 -1.62005756509237e-13 -5.76991542573971 -24.5334169783283;-6e-05 -1.56982290659279e-13 -5.19331649259106 -24.7346720555941]  x2=[-0.00066 -1.35923509993764e-14 0 0;-0.0006 -1.34631382189715e-14 0 0;-0.00054 -1.33270374482836e-14 0 0;-0.00048 -1.31841183189818e-14 0 0;-0.00042 -1.30344539511335e-14 -0.00037674948649764 -0.0129346292684651;-0.00036 -1.28781209157948e-14 -7.76188242684462e-05 -0.0129582402107961;-0.0003 -1.27151991958353e-14 0.000221551549185474 -0.0129752214779945;-0.00024 -1.25457721450173e-14 0.00052060857277303 -0.0129855643821302;-0.00018 -1.23699264453507e-14 0.000819399243395014 -0.0129892636315824;-0.00012 -1.21877520627447e-14 0.00111777069422332 -0.0129863173337467;-6e-05 -1.19993422009796e-14 0.00141557027291043 -0.0129767269960034]  x3=[-0.00066 4.73623718829333e-15 0 0;-0.0006 4.86790625194776e-15 0 0;-0.00054 4.99708480481513e-15 0 0;-0.00048 5.12370675676084e-15 0 0;-0.00042 5.24770732565458e-15 3.59452843596048 -2.19161260421971;-0.00036 5.36902307051404e-15 3.63237824754622 -2.11535545563163;-0.0003 5.48759192396248e-15 3.66836966730188 -2.03801605210518;-0.00024 5.60335322398358e-15 3.70248428135208 -1.95963396190827;-0.00018 5.71624774495722e-15 3.73470463602989 -1.88024928676657;-0.00012 5.82621772796044e-15 3.7650142468065 -1.79990264134675;-6e-05 5.9332069103179e-15 3.79339760672498 -1.71863513247724]  x4=[-0.00066 -7.14795217667827e-15 0 0;-0.0006 -7.242547776064e-15 0 0;-0.00054 -7.33343795418059e-15 0 0;-0.00048 -7.42057620993347e-15 0 0;-0.00042 -7.50391796178087e-15 -3.82381011037688 1.69503190262537;-0.00036 -7.58342057054255e-15 -3.84961517563703 1.61212236693045;-0.0003 -7.65904336121485e-15 -3.87345070664061 1.52838803964401;-0.00024 -7.7307476437807e-15 -3.89530450868954 1.44387176079512;-0.00018 -7.7984967330042e-15 -3.91516540097487 1.35861677047373;-0.00012 -7.86225596719944e-15 -3.93302322229712 1.27266668670821;-6e-05 -7.92199272596408e-15 -3.94886883626493 1.1860654831496]  x5=0.000627751139365274  V1=[1.134e-27 1.175e-15 1.175e-15;377 377 377;0.8883 -1.731 2.981]  V2=[1.245e-23 7.93e-13 7.93e-13;377 377 377;-1.459 -1.742 2.971]  I1=[6.861e-26 2.027e-14 2.027e-14;377 377 377;-2.79 3.007 1.436]  I2=[6.467e-26 2.017e-14 2.017e-14;377 377 377;0.1116 -0.2797 -1.851]  nHarmo=1  Measurements=None  Decoupling=off  VsMag0=0  VrMag0=0  VsAngle0=0  VrAngle0=0  IsMag0=0  IrMag0=0  IsAngle0=0  IrAngle0=0
      settings: LibrarySourceBlock=sps_lib/Power Grid Elements/Distributed Parameters Line
  MPP3_800MVA 17KV : spsSynchronousMachinepuStandardLib/Synchronous Machine pu Standard  PresetModel=No  MechanicalLoad=Mechanical power Pm  ShowDetailedParameters=on  RotorType=Salient-pole  Units=per unit standard parameters  MeasurementBus=off  NominalParameters=[800e6 17000 60]  Reactances1=[ 1.81, 0.3, 0.23, 1.76, 0.65, 0.25, 0.15 ]  Reactances2=[2.24 0.17 0.12 1.02 0.13 0.08]  dAxisTimeConstants=Short-circuit  qAxisTimeConstants=Open-circuit  TimeConstants1="[ 4.4849  0.0681  0.1  ]"  TimeConstants2=[ 8.0, 0.03, 1.0, 0.07 ]  TimeConstants3="[  4.49  0.0681  0.0513  ]"  TimeConstants4=[ 8.0, 0.03, 0.3371, 0.0295 ]  TimeConstants5=[ 1.01, 0.053, 0.1 ]  TimeConstants6=[ 1.3201, 0.023, 1.0, 0.07 ]  TimeConstants7=[0.012 0.003 0.003]  TimeConstants8=[ 1.3201, 0.0231, 0.3371, 0.0295 ]  StatorResistance=0.037875  Mechanical=[3.8 0 28]  PolePairs=20  InitialConditions="[  0 -94.876 0.604539 0.604539 0.604539 -42.1129 -162.113 77.8871 1.28555 ]"  SetSaturation=off  Saturation=[0.6404,0.7127,0.8441,0.9214,0.9956,1.082,1.19,1.316,1.457;0.7,0.7698,0.8872,0.9466,0.9969,1.046,1.1,1.151,1.201]  LoadFlowParameters=[1,0,0,0,0]  TsPowergui=0  TsBlock=-1  IterativeModel=Trapezoidal non iterative  IterativeDiscreteModel=Trapezoidal non iterative  BusType=PV  Pref=500e6  Qref=0  Qmin=-inf  Qmax=inf  PLF=0  QLF=0
  MPP4-TEST2 96 km : spsDistributedParametersLineLib/Distributed Parameters Line  Phases=3  Length=96  Frequency=60  Resistance=[0.01273 0.3864]/6  Inductance="[0.9337e-3  4.1264e-3]/6"  Capacitance=[12.74e-9 7.751e-9]*6  x1=[-0.0006 -4.5857760226163e-15 2.37990855723243 -27.6655669674231;-0.00054 -1.80503612714193e-15 3.00502751630967 -27.6046611878373;-0.00048 9.7662725816831e-16 3.62860904778304 -27.5296323535123;-0.00042 3.75779098292728e-15 4.25033411581858 -27.4405188505861;-0.00036 6.53703215238339e-15 4.86988463438332 -27.3373662711735;-0.0003 9.31292885539988e-15 5.48694362998399 -27.2202273900401;-0.00024 1.20840608919308e-14 6.10119540383649 -27.089162137602;-0.00018 1.48490104996216e-14 6.71232569338327 -26.9442375692641;-0.00012 1.76063630791627e-14 7.32002183307579 -26.7855278311135;-6e-05 2.03547079180243e-14 7.92397291434006 -26.6131141219849]  x2=[-0.0006 -1.34631382189715e-14 -0.00127237336942136 -0.0128241561091282;-0.00054 -1.33270374482836e-14 -0.00097427961280095 -0.0128675700632669;-0.00048 -1.31841183189818e-14 -0.000675687396728012 -0.0129044007307959;-0.00042 -1.30344539511335e-14 -0.00037674948649764 -0.0129346292684651;-0.00036 -1.28781209157948e-14 -7.76188242684462e-05 -0.0129582402107961;-0.0003 -1.27151991958353e-14 0.000221551549185474 -0.0129752214779945;-0.00024 -1.25457721450173e-14 0.00052060857277303 -0.0129855643821302;-0.00018 -1.23699264453507e-14 0.000819399243395014 -0.0129892636315824;-0.00012 -1.21877520627447e-14 0.00111777069422332 -0.0129863173337467;-6e-05 -1.19993422009796e-14 0.00141557027291043 -0.0129767269960034]  x3=[-0.0006 3.89432093218755e-15 4.90431800617941 -0.0150079232796438;-0.00054 3.90354678700557e-15 4.90340629357799 0.095920656025339;-0.00048 3.9107755151581e-15 4.89998590771225 0.206800160550289;-0.00042 3.91600341829426e-15 4.89405859851479 0.317573862291874;-0.00036 3.91922782172219e-15 4.88562739850652 0.428185087377421;-0.0003 3.92044707577753e-15 4.87469662124517 0.538577245060314;-0.00024 3.91966055666736e-15 4.86127185911834 0.648693856672871;-0.00018 3.91686866678941e-15 4.84535998048242 0.75847858452187;-0.00012 3.91207283452611e-15 4.82696912614853 0.867875260711955;-6e-05 3.90527551351388e-15 4.80610870521756 0.976827915882169]  x4=[-0.0006 -3.86079222720682e-15 -4.8900275552317 -0.599643853074957;-0.00054 -3.82965996936989e-15 -4.8752173779525 -0.710092345945148;-0.00048 -3.79656838672865e-15 -4.85791294937909 -0.820177542450156;-0.00042 -3.76153440954824e-15 -4.83812312277686 -0.929843120969308;-0.00036 -3.72457596185875e-15 -4.81585802298679 -1.03903297456625;-0.0003 -3.68571195228491e-15 -4.79112904124533 -1.14769123969428;-0.00024 -3.64496226437216e-15 -4.76394882935648 -1.25576232477718;-0.00018 -3.6023477464138e-15 -4.73433129321888 -1.36319093865091;-0.00012 -3.55789020078464e-15 -4.70229158571129 -1.46992211885155;-6e-05 -3.51161237278651e-15 -4.66784609894008 -1.57590125973515]  x5=0.000542919904315913  V1=[8.106e-27 2.861e-16 2.861e-16;377 377 377;-1.836 -1.712 3.001]  V2=[1.245e-23 7.93e-13 7.93e-13;377 377 377;-1.427 -1.722 2.99]  I1=[7.942e-26 2.345e-14 2.345e-14;377 377 377;-2.756 3.026 1.455]  I2=[7.544e-26 2.335e-14 2.335e-14;377 377 377;0.1775 -0.2404 -1.811]  nHarmo=1  Measurements=None  Decoupling=off  VsMag0=0  VrMag0=0  VsAngle0=0  VrAngle0=0  IsMag0=0  IrMag0=0  IsAngle0=0  IrAngle0=0
      settings: LibrarySourceBlock=sps_lib/Power Grid Elements/Distributed Parameters Line
  MPP4_3800MVA 17KV : spsSynchronousMachinepuStandardLib/Synchronous Machine pu Standard  PresetModel=No  MechanicalLoad=Mechanical power Pm  ShowDetailedParameters=on  RotorType=Salient-pole  Units=per unit standard parameters  MeasurementBus=off  NominalParameters=[3800e6 17000 60]  Reactances1=[ 1.81, 0.3, 0.23, 1.76, 0.65, 0.25, 0.15 ]  Reactances2=[2.24 0.17 0.12 1.02 0.13 0.08]  dAxisTimeConstants=Short-circuit  qAxisTimeConstants=Open-circuit  TimeConstants1="[ 4.4849  0.0681  0.1  ]"  TimeConstants2=[ 8.0, 0.03, 1.0, 0.07 ]  TimeConstants3="[  4.49  0.0681  0.0513  ]"  TimeConstants4=[ 8.0, 0.03, 0.3371, 0.0295 ]  TimeConstants5=[ 1.01, 0.053, 0.1 ]  TimeConstants6=[ 1.3201, 0.023, 1.0, 0.07 ]  TimeConstants7=[0.012 0.003 0.003]  TimeConstants8=[ 1.3201, 0.0231, 0.3371, 0.0295 ]  StatorResistance=0.037875  Mechanical=[3.8 0 28]  PolePairs=20  InitialConditions=[ 0 -113.876 0.904539 0.904539 0.904539 -42.1129 -162.113 77.8871 1.28555]  SetSaturation=off  Saturation=[0.6404,0.7127,0.8441,0.9214,0.9956,1.082,1.19,1.316,1.457;0.7,0.7698,0.8872,0.9466,0.9969,1.046,1.1,1.151,1.201]  LoadFlowParameters=[1,0,0,0,0]  TsPowergui=0  TsBlock=-1  IterativeModel=Trapezoidal non iterative  IterativeDiscreteModel=Trapezoidal non iterative  BusType=PV  Pref=3200e6  Qref=0  Qmin=-inf  Qmax=inf  PLF=0  QLF=0
  MPP5_4200MVA 17KV : spsSynchronousMachinepuStandardLib/Synchronous Machine pu Standard  PresetModel=No  MechanicalLoad=Mechanical power Pm  ShowDetailedParameters=on  RotorType=Salient-pole  Units=per unit standard parameters  MeasurementBus=off  NominalParameters=[4200e6 17000 60]  Reactances1=[ 1.81, 0.3, 0.23, 1.76, 0.65, 0.25, 0.15 ]  Reactances2=[2.24 0.17 0.12 1.02 0.13 0.08]  dAxisTimeConstants=Short-circuit  qAxisTimeConstants=Open-circuit  TimeConstants1="[ 4.4849  0.0681  0.1  ]"  TimeConstants2=[ 8.0, 0.03, 1.0, 0.07 ]  TimeConstants3="[  4.49  0.0681  0.0513  ]"  TimeConstants4=[ 8.0, 0.03, 0.3371, 0.0295 ]  TimeConstants5=[ 1.01, 0.053, 0.1 ]  TimeConstants6=[ 1.3201, 0.023, 1.0, 0.07 ]  TimeConstants7=[0.012 0.003 0.003]  TimeConstants8=[ 1.3201, 0.0231, 0.3371, 0.0295 ]  StatorResistance=0.037875  Mechanical=[3.8 0 28]  PolePairs=20  InitialConditions="[  0 -73.876 0.604539 0.604539 0.604539 -42.1129 -162.113 77.8871 1.28555]"  SetSaturation=off  Saturation=[0.6404,0.7127,0.8441,0.9214,0.9956,1.082,1.19,1.316,1.457;0.7,0.7698,0.8872,0.9466,0.9969,1.046,1.1,1.151,1.201]  LoadFlowParameters=[1,0,0,0,0]  TsPowergui=0  TsBlock=-1  IterativeModel=Trapezoidal non iterative  IterativeDiscreteModel=Trapezoidal non iterative  BusType=PV  Pref=3200e6  Qref=0  Qmin=-inf  Qmax=inf  PLF=0  QLF=0
  MPP6-CSG 186 km : spsDistributedParametersLineLib/Distributed Parameters Line  Phases=3  Length=186  Frequency=60  Resistance=[0.01273 0.3864]/6  Inductance="[0.9337e-3  4.1264e-3]/6"  Capacitance=[12.74e-9 7.751e-9]*6  x1=[-0.00108 -3.07956012617368e-12 0 0;-0.00102 -3.06961927236044e-12 0 0;-0.00096 -3.05810794460741e-12 0 0;-0.0009 -3.04503203232258e-12 0 0;-0.00084 -3.0303982253843e-12 0 0;-0.00078 -3.01421401071858e-12 0 0;-0.00072 -2.99648766846872e-12 0 0;-0.00066 -2.97722826775894e-12 0.0652053953357076 -0.103488683577159;-0.0006 -2.95644566205451e-12 0.0680082277148552 -0.102742369381794;-0.00054 -2.93415048412055e-12 0.0707762658280562 -0.101943490291793;-0.00048 -2.91035414058205e-12 0.0735080934958647 -0.10109245502846;-0.00042 -2.88506880608806e-12 0.0762023130647672 -0.10018969899716;-0.00036 -2.85830741708293e-12 0.078857546122249 -0.0992356840645602;-0.0003 -2.83008366518778e-12 0.0814724342020147 -0.0982308983223286;-0.00024 -2.80041199019558e-12 0.0840456394790051 -0.0971758558374169;-0.00018 -2.76930757268354e-12 0.0865758454538532 -0.0960710963890555;-0.00012 -2.73678632624638e-12 0.0890617576264295 -0.0949171851925918;-6e-05 -2.70286488935473e-12 0.091502104158132 -0.0937147126103155]  x2=[-0.00108 -3.42305362207819e-12 0 0;-0.00102 -3.34365772116779e-12 0 0;-0.00096 -3.26255114318354e-12 0 0;-0.0009 -3.17977538374943e-12 0 0;-0.00084 -3.0953727924735e-12 0 0;-0.00078 -3.00938655128102e-12 0 0;-0.00072 -2.92186065232185e-12 0 0;-0.00066 -2.83283987546316e-12 1.06374283647725 -1.39266589939745;-0.0006 -2.74236976537933e-12 1.10710669036806 -1.38836686006487;-0.00054 -2.65049660825036e-12 1.1499041280191 -1.38335750659262;-0.00048 -2.55726740808106e-12 1.19211325347045 -1.37764040185848;-0.00042 -2.46272986265292e-12 1.23371247175361 -1.37121847083889;-0.00036 -2.36693233912104e-12 1.27468049993984 -1.36409499911241;-0.0003 -2.26992384926857e-12 1.31499637802891 -1.35627363117881;-0.00024 -2.17175402443146e-12 1.35463947967264 -1.34775836859444;-0.00018 -2.07247309010604e-12 1.39358952272771 -1.33855356792498;-0.00012 -1.97213184025282e-12 1.43182657963238 -1.32866393851655;-6e-05 -1.87078161130932e-12 1.4693310876018 -1.31809454008629]  x3=[-0.00108 -8.43749804415317e-14 0 0;-0.00102 -8.42236158997915e-14 0 0;-0.00096 -8.40291609998835e-14 0 0;-0.0009 -8.37917152285277e-14 0 0;-0.00084 -8.3511400067368e-14 0 0;-0.00078 -8.31883589308206e-14 0 0;-0.00072 -8.28227570927001e-14 0 0;-0.00066 -8.24147816016623e-14 -0.161678982528037 -0.0197142925397632;-0.0006 -8.19646411855071e-14 -0.159359196790469 -0.0223722030080845;-0.00054 -8.14725661443889e-14 -0.156957879943204 -0.0250186674439562;-0.00048 -8.09388082329913e-14 -0.154476260544312 -0.0276523318672716;-0.00042 -8.03636405317246e-14 -0.151915608236132 -0.0302718488466475;-0.00036 -7.97473573070124e-14 -0.1492772330957 -0.0328758781887939;-0.0003 -7.90902738607403e-14 -0.146562484964491 -0.0354630876241826;-0.00024 -7.83927263689407e-14 -0.143772752757811 -0.0380321534886602;-0.00018 -7.76550717097998e-14 -0.140909463754205 -0.0405817614006596;-0.00012 -7.68776872810714e-14 -0.137974082865234 -0.0431106069336617;-6e-05 -7.60609708069936e-14 -0.134968111886002 -0.0456173962835642]  x4=[-0.00108 2.86482923275602e-14 0 0;-0.00102 2.89493523707862e-14 0 0;-0.00096 2.92356013904167e-14 0 0;-0.0009 2.95068929361642e-14 0 0;-0.00084 2.97630882102607e-14 0 0;-0.00078 3.00040561384703e-14 0 0;-0.00072 3.02296734371483e-14 0 0;-0.00066 3.04398246763156e-14 0.181028281864538 -0.0137802447017299;-0.0006 3.06344023387152e-14 0.179794852281121 -0.0111018424840778;-0.00054 3.08133068748197e-14 0.178469436329049 -0.00841776035867245;-0.00048 3.09764467537626e-14 0.177052712115616 -0.00572937155152523;-0.00042 3.11237385101673e-14 0.175545404463106 -0.00303805149202563;-0.00036 3.12551067868497e-14 0.173948284537967 -0.00034517710924598;-0.0003 3.1370484373372e-14 0.172262169456264 0.0023478738725209;-0.00024 3.14698122404289e-14 0.170487921865627 0.00503972363863088;-0.00018 3.15530395700483e-14 0.16862644950391 0.00772899498900395;-0.00012 3.16201237815906e-14 0.166678704734768 0.0104143120427252;-6e-05 3.16710305535335e-14 0.164645684060415 0.0130943009419711]  x5=0.00105190731461208  V1=[8.574e-27 4.511e-17 4.511e-17;377 377 377;-2.265 1.301 -0.2697]  V2=[1.073e-22 6.76e-12 6.76e-12;377 377 377;0.1921 1.269 -0.3021]  I1=[3.519e-25 1.037e-13 1.037e-13;377 377 377;-1.143 -0.2664 -1.837]  I2=[3.187e-25 1.028e-13 1.028e-13;377 377 377;1.591 2.633 1.062]  nHarmo=1  Measurements=None  Decoupling=off  VsMag0=0  VrMag0=0  VsAngle0=0  VrAngle0=0  IsMag0=0  IrMag0=0  IsAngle0=0  IrAngle0=0
      settings: LibrarySourceBlock=sps_lib/Power Grid Elements/Distributed Parameters Line
  MPP6_490MVA 17KV : spsSynchronousMachinepuStandardLib/Synchronous Machine pu Standard  PresetModel=No  MechanicalLoad=Mechanical power Pm  ShowDetailedParameters=on  RotorType=Salient-pole  Units=per unit standard parameters  MeasurementBus=off  NominalParameters=[490e6 13800 60]  Reactances1=[ 1.81, 0.3, 0.23, 1.76, 0.65, 0.25, 0.15 ]  Reactances2=[2.24 0.17 0.12 1.02 0.13 0.08]  dAxisTimeConstants=Short-circuit  qAxisTimeConstants=Open-circuit  TimeConstants1="[ 4.4849  0.0681  0.1  ]"  TimeConstants2=[ 8.0, 0.03, 1.0, 0.07 ]  TimeConstants3="[  4.49  0.0681  0.0513  ]"  TimeConstants4=[ 8.0, 0.03, 0.3371, 0.0295 ]  TimeConstants5=[ 1.01, 0.053, 0.1 ]  TimeConstants6=[ 1.3201, 0.023, 1.0, 0.07 ]  TimeConstants7=[0.012 0.003 0.003]  TimeConstants8=[ 1.3201, 0.0231, 0.3371, 0.0295 ]  StatorResistance=0.037875  Mechanical=[3.8 0 28]  PolePairs=20  InitialConditions="[  0 -76.876 0.604539 0.604539 0.604539 -42.1129 -162.113 77.8871 1.28555]"  SetSaturation=off  Saturation=[0.6404,0.7127,0.8441,0.9214,0.9956,1.082,1.19,1.316,1.457;0.7,0.7698,0.8872,0.9466,0.9969,1.046,1.1,1.151,1.201]  LoadFlowParameters=[1,0,0,0,0]  TsPowergui=0  TsBlock=-1  IterativeModel=Trapezoidal non iterative  IterativeDiscreteModel=Trapezoidal non iterative  BusType=PV  Pref=350e6  Qref=0  Qmin=-inf  Qmax=inf  PLF=0  QLF=0
  PNS-CON 260 km : spsDistributedParametersLineLib/Distributed Parameters Line  Phases=3  Length=271  Frequency=60  Resistance=[0.01273 0.3864]/6  Inductance="[0.9337e-3  4.1264e-3]/6"  Capacitance=[12.74e-9 7.751e-9]*6  x1=[-0.00156 6.04527781172368e-15 -0.000796952505926034 0.00149346225128385;-0.0015 5.94176846161128e-15 -0.000834728778609639 0.00148194376506084;-0.00144 5.83521919296265e-15 -0.000872077988626094 0.00146966708902445;-0.00138 5.72568451835246e-15 -0.000908981027429418 0.00145663850414899;-0.00132 5.61322047774419e-15 -0.000945419014743071 0.00144286467609923;-0.00126 5.49788460981911e-15 -0.000981373308219447 0.0014283526518201;-0.0012 5.37973592253843e-15 -0.00101682551297764 0.00141310985593137;-0.00114 5.25883486295368e-15 -0.00105175749101463 0.00139714408692908;-0.00108 5.13524328628095e-15 -0.00108615137048496 0.00138046351319567;-0.00102 5.00902442425458e-15 -0.00111998955484439 0.00136307666882087;-0.00096 4.88024285277663e-15 -0.00115325473185253 0.00134499244923554;-0.0009 4.74896445887867e-15 -0.00118592988243016 0.00132622010666058;-0.00084 4.61525640701278e-15 -0.00121799828936647 0.00130676924537332;-0.00078 4.47918710468893e-15 -0.00124944354587192 0.00128664981679381;-0.00072 4.34082616747646e-15 -0.00128024956397224 0.00126587211439347;-0.00066 4.20024438338746e-15 -0.00131040058273934 0.00124444676842878;-0.0006 4.05751367666033e-15 -0.00133988117635489 0.00122238474050263;-0.00054 3.91270707096199e-15 -0.00136867626200246 0.00119969731795617;-0.00048 3.76589865202763e-15 -0.00139677110758416 0.00117639610809398;-0.00042 3.61716352975708e-15 -0.00142415133925786 0.00115249303224559;-0.00036 3.46657779978722e-15 -0.0014508029487911 0.00112800031966628;-0.0003 3.31421850455999e-15 -0.00147671230072798 0.00110293050128038;-0.00024 3.16016359390611e-15 -0.00150186613936531 0.00107729640327022;-0.00018 3.00449188516448e-15 -0.00152625159553444 0.00105111114051399;-0.00012 2.84728302285777e-15 -0.00154985619318541 0.00102438810987597;-6e-05 2.68861743794483e-15 -0.0015726678557699 0.000997140983352427]  x2=[-0.00156 -5.47744132593486e-12 -5.87038523997561 7.29063222176106;-0.0015 -5.40246500229258e-12 -6.08013946822921 7.22558203662831;-0.00144 -5.32472467772906e-12 -6.28678298478282 7.1568351102122;-0.00138 -5.24426012563081e-12 -6.49021006699501 7.08442661471061;-0.00132 -5.16111251314951e-12 -6.69031663781163 7.00839359564778;-0.00126 -5.07532438014008e-12 -6.88700031901351 6.92877495292119;-0.0012 -4.98693961739656e-12 -7.08016048359505 6.84561142089964;-0.00114 -4.89600344419673e-12 -7.26969830724686 6.75894554758281;-0.00108 -4.80256238516711e-12 -7.4555168189161 6.66882167283288;-0.00102 -4.70666424648008e-12 -7.63752095041867 6.57528590568947;-0.00096 -4.6083580913954e-12 -7.81561758507785 6.4783861007794;-0.0009 -4.5076942151585e-12 -7.98971560536449 6.37817183383336;-0.00084 -4.40472411926851e-12 -8.15972593951446 6.27469437632206;-0.00078 -4.29950048512916e-12 -8.32556160709938 6.16800666922482;-0.00072 -4.19207714709598e-12 -8.48713776352741 6.05816329594394;-0.00066 -4.08250906493367e-12 -8.64437174345134 5.94522045437886;-0.0006 -3.97085229569764e-12 -8.7971831030617 5.82923592817429;-0.00054 -3.85716396505422e-12 -8.94549366124329 5.71026905715697;-0.00048 -3.74150223805408e-12 -9.08922753957406 5.58838070697636;-0.00042 -3.62392628937395e-12 -9.22831120114597 5.46363323796466;-0.00036 -3.50449627304171e-12 -9.36267348818779 5.33609047323209;-0.0003 -3.38327329166053e-12 -9.49224565847074 5.20581766601379;-0.00024 -3.26031936514764e-12 -9.61696142047828 5.07288146628511;-0.00018 -3.13569739900377e-12 -9.73675696732208 4.93734988666221;-0.00012 -3.00947115212954e-12 -9.85157100938683 4.79929226760556;-6e-05 -2.88170520420524e-12 -9.96134480568707 4.65877924194407]  x3=[-0.00156 -5.98908273642193e-14 0.581974611890026 0.194405948890548;-0.0015 -6.12942242928234e-14 0.572890091039119 0.204721101522632;-0.00144 -6.26662619636922e-14 0.563512469031845 0.214931515056367;-0.00138 -6.40062384170009e-14 0.553846543632902 0.225031965655521;-0.00132 -6.53134680960363e-14 0.543897260108328 0.235017285742933;-0.00126 -6.65872821979395e-14 0.533669708695416 0.244882366644339;-0.0012 -6.78270290158788e-14 0.523169121998454 0.254622161202063;-0.00114 -6.90320742724742e-14 0.512400872311624 0.26423168635724;-0.00108 -7.02018014443057e-14 0.501370468870439 0.273706025699237;-0.00102 -7.13356120773381e-14 0.490083555033119 0.28304033198098;-0.00096 -7.24329260931013e-14 0.478545905393341 0.292229829598897;-0.0009 -7.34931820854686e-14 0.466763422825853 0.301269817036206;-0.00084 -7.45158376078831e-14 0.45474213546645 0.310155669268292;-0.00078 -7.55003694508831e-14 0.442488193627874 0.318882840128963;-0.00072 -7.64462739097855e-14 0.430007866653197 0.327446864636346;-0.00066 -7.7353067042391e-14 0.417307539708308 0.33584336127726;-0.0006 -7.82202849165773e-14 0.404393710515147 0.344068034248872;-0.00054 -7.90474838476556e-14 0.39127298602735 0.352116675656516;-0.00048 -7.98342406253678e-14 0.377952079050008 0.359985167666526;-0.00042 -8.05801527304089e-14 0.364437804805272 0.367669484612996;-0.00036 -8.12848385403632e-14 0.350737077445562 0.375165695057388;-0.0003 -8.1947937524949e-14 0.336856906516155 0.382469963799923;-0.00024 -8.25691104304734e-14 0.322804393368974 0.389578553841746;-0.00018 -8.31480394533997e-14 0.308586727529406 0.39648782829684;-0.00012 -8.36844284029426e-14 0.294211183018007 0.403194252252724;-6e-05 -8.4178002852604e-14 0.279685114628978 0.409694394578982]  x4=[-0.00156 1.22010463566512e-14 -0.674222424971416 -0.0233872640497449;-0.0015 1.38777541429234e-14 -0.670272883538504 -0.0344867199253624;-0.00144 1.55473618137447e-14 -0.665980418113155 -0.0455685317578249;-0.00138 1.72090151669798e-14 -0.661347224799995 -0.0566270298874303;-0.00132 1.88618640700695e-14 -0.656375674026337 -0.0676565565821981;-0.00126 2.05050628949737e-14 -0.651068309329418 -0.078651468932469;-0.0012 2.21377709508109e-14 -0.645427846055088 -0.0896061417379221;-0.00114 2.37591529139707e-14 -0.63945716996858 -0.100514970385531;-0.00108 2.5368379255481e-14 -0.633159335778107 -0.111372373716987;-0.00102 2.69646266654104e-14 -0.62653756557201 -0.122172796884125;-0.00096 2.85470784740889e-14 -0.619595247170283 -0.132910714190884;-0.0009 3.01149250699306e-14 -0.6123359323913 -0.143580631920354;-0.00084 3.16673643136467e-14 -0.604763335234639 -0.154177091145469;-0.00078 3.32036019486343e-14 -0.59688132998093 -0.16469467052189;-0.00072 3.4722852007333e-14 -0.588693949209704 -0.175127989061663;-0.00066 3.62243372133402e-14 -0.580205381736248 -0.185471708886239;-0.0006 3.77072893790802e-14 -0.571419970468534 -0.195720537957426;-0.00054 3.91709497988234e-14 -0.562342210185301 -0.205869232784895;-0.00048 4.06145696368535e-14 -0.552976745236448 -0.215912601108844;-0.00042 4.20374103105864e-14 -0.543328367166896 -0.22584550455646;-0.00036 4.34387438684424e-14 -0.533402012265148 -0.2356628612708;-0.0003 4.48178533622796e-14 -0.523202759037789 -0.245359648510764;-0.00024 4.6174033214198e-14 -0.512735825611231 -0.254930905220826;-0.00018 4.75065895775259e-14 -0.502006567062022 -0.264371734569195;-0.00012 4.88148406918052e-14 -0.491020472677088 -0.273677306453131;-6e-05 5.00981172315919e-14 -0.479783163145318 -0.282842859970109]  x5=0.00153261764655846  V1=[1.516e-17 3.586e-06 3.586e-06;377 377 377;3.054 -1.986 2.727]  V2=[2.167e-13 0.2213 0.2213;377 377 377;-0.8435 -2.017 2.695]  I1=[4.914e-16 0.002352 0.002352;377 377 377;-2.188 2.73 1.159]  I2=[4.262e-16 0.002322 0.002322;377 377 377;0.3532 -0.7649 -2.336]  nHarmo=1  Measurements=None  Decoupling=off  VsMag0=0  VrMag0=0  VsAngle0=0  VrAngle0=0  IsMag0=0  IrMag0=0  IsAngle0=0  IrAngle0=0
      settings: LibrarySourceBlock=sps_lib/Power Grid Elements/Distributed Parameters Line
  PNS3 : spsThreePhaseVIMeasurementLib/Three-Phase V-I Measurement  VoltageMeasurement=no  SetLabelV=off  LabelV=Vabc  Vpu=off  VpuLL=off  CurrentMeasurement=no  SetLabelI=off  LabelI=Iabc  Ipu=off  Pbase=100e6  Vbase=500e3  OutputType=Complex  PhasorSimulation=off  PSBequivalent=0
  Regulators 1 : Subsystem
  Regulators 2 : Subsystem
  Regulators 3 : Subsystem
  Regulators 4 : Subsystem
  Regulators 5 : Subsystem
  Regulators 6 : Subsystem
  TEST 1 : spsThreePhaseVIMeasurementLib/Three-Phase V-I Measurement  VoltageMeasurement=no  SetLabelV=off  LabelV=Vabc  Vpu=off  VpuLL=off  CurrentMeasurement=no  SetLabelI=off  LabelI=Iabc  Ipu=off  Pbase=100e6  Vbase=500e3  OutputType=Complex  PhasorSimulation=off  PSBequivalent=0
  TEST1-MPP2 187 km : spsDistributedParametersLineLib/Distributed Parameters Line  Phases=3  Length=187  Frequency=60  Resistance=[0.01273 0.3864]/6  Inductance="[0.9337e-3  4.1264e-3]/6"  Capacitance=[12.74e-9 7.751e-9]*6  x1=[-0.00108 2.13973803419253e-12 0 0;-0.00102 2.10318394336915e-12 0 0;-0.00096 2.06555382477797e-12 0 0;-0.0009 2.02686693068299e-12 0 0;-0.00084 1.98714305401407e-12 0 0;-0.00078 1.94640251824054e-12 0 0;-0.00072 1.9046661669733e-12 0 0;-0.00066 1.86195535330085e-12 0.190167453671412 0.0876837438700702;-0.0006 1.81829192886466e-12 0.192515613369267 0.0831662011860424;-0.00054 1.7736982326795e-12 0.194765278522042 0.0786061091367531;-0.00048 1.72819707970433e-12 0.196915298159477 0.0740058007495555;-0.00042 1.68181174916977e-12 0.198964572291797 0.0693676296272245;-0.00036 1.63456597266803e-12 0.200912052472491 0.0646939687438098;-0.0003 1.58648392201136e-12 0.202756742334711 0.0599872092305786;-0.00024 1.53759019686534e-12 0.204497698101039 0.0552497591526689;-0.00018 1.4879098121632e-12 0.206134029066335 0.0504840422770785;-0.00012 1.43746818530775e-12 0.207664898053443 0.0456924968326214;-6e-05 1.38629112316733e-12 0.2090895218415 0.0408775742624843]  x2=[-0.00108 -1.76998250026953e-12 0 0;-0.00102 -1.77357329527998e-12 0 0;-0.00096 -1.7762566974207e-12 0 0;-0.0009 -1.77803133381356e-12 0 0;-0.00084 -1.77889629652181e-12 0 0;-0.00078 -1.77885114301453e-12 0 0;-0.00072 -1.7778958963931e-12 0 0;-0.00066 -1.77603104537933e-12 -1.8495779026508 -0.154143455225187;-0.0006 -1.77325754406547e-12 -1.85243672391596 -0.112397108416225;-0.00054 -1.76957681142603e-12 -1.85434780432407 -0.0705932571697387;-0.00048 -1.76499073059184e-12 -1.85531016613108 -0.0287532891084704;-0.00042 -1.75950164788661e-12 -1.85532331697491 0.0131013896668054;-0.00036 -1.75311237162646e-12 -1.85438725012734 0.0549493655290419;-0.0003 -1.7458261706832e-12 -1.85250244449747 0.0967692282805261;-0.00024 -1.73764677281185e-12 -1.84966986438668 0.138539582106732;-0.00018 -1.72857836274352e-12 -1.84589095899531 0.180239056522816;-0.00012 -1.71862558004435e-12 -1.84116766168117 0.221846317307147;-6e-05 -1.70779351674188e-12 -1.83550238897045 0.263340077416295]  x3=[-0.00108 -2.58778747599844e-14 0 0;-0.00102 -2.7606089157311e-14 0 0;-0.00096 -2.93201797693228e-14 0 0;-0.0009 -3.10192696355899e-14 0 0;-0.00084 -3.27024894703413e-14 0 0;-0.00078 -3.43689781072072e-14 0 0;-0.00072 -3.60178829398077e-14 0 0;-0.00066 -3.76483603579623e-14 0.0204172813974424 -0.185308577335573;-0.0006 -3.9259576179296e-14 0.0162347958571241 -0.185704397345926;-0.00054 -4.08507060760228e-14 0.0120440042952608 -0.186005207555173;-0.00048 -4.24209359966868e-14 0.00784705079825244 -0.186210854063254;-0.00042 -4.39694625826462e-14 0.00364608260505886 -0.186321231657615;-0.00036 -4.54954935790861e-14 -0.000556750991367331 -0.18633628386704;-0.0003 -4.69982482403508e-14 -0.00475929974369876 -0.18625600299054;-0.00024 -4.8476957729388e-14 -0.00895941355033957 -0.186080430101294;-0.00018 -4.99308655110996e-14 -0.0131549435554571 -0.185809655025638;-0.00012 -5.13592277393995e-14 -0.0173437432483762 -0.185443816297103;-6e-05 -5.27613136377784e-14 -0.021523669561774 -0.184983101085543]  x4=[-0.00108 3.14995876161522e-14 0 0;-0.00102 3.29345406091501e-14 0 0;-0.00096 3.4352643682612e-14 0 0;-0.0009 3.5753171308802e-14 0 0;-0.00084 3.71354069519078e-14 0 0;-0.00078 3.84986434346335e-14 0 0;-0.00072 3.9842183300005e-14 0 0;-0.00066 4.11653391682012e-14 -0.0568407827484481 0.179409909103137;-0.0006 4.2467434088231e-14 -0.0527707501292256 0.180622471855651;-0.00054 4.37478018842733e-14 -0.0486737190191457 0.181742624814045;-0.00048 4.50057874965052e-14 -0.0445517855350287 0.182769794887366;-0.00042 4.62407473162425e-14 -0.0404070585342096 0.183703456556426;-0.00036 4.74520495152221e-14 -0.0362416585356079 0.184543132142661;-0.0003 4.86390743688566e-14 -0.0320577166348304 0.185288392052527;-0.00024 4.98012145732973e-14 -0.0278573734138641 0.185938854997284;-0.00018 5.09378755561416e-14 -0.0236427778459142 0.186494188188069;-0.00012 5.20484757806277e-14 -0.01941608619595 0.18695410750616;-6e-05 5.31324470431591e-14 -0.0151794609175199 0.187318377648337]  x5=0.00105756273028204  V1=[5.148e-22 3.64e-12 3.64e-12;377 377 377;-2.284 2.392 -2.32]  V2=[4.457e-19 3.159e-07 3.159e-07;377 377 377;1.876 2.36 -2.352]  I1=[1.453e-21 4.823e-09 4.823e-09;377 377 377;0.5394 0.8251 2.396]  I2=[1.317e-21 4.781e-09 4.781e-09;377 377 377;-3.011 -2.56 -0.9894]  nHarmo=1  Measurements=None  Decoupling=off  VsMag0=0  VrMag0=0  VsAngle0=0  VrAngle0=0  IsMag0=0  IrMag0=0  IsAngle0=0  IrAngle0=0
      settings: LibrarySourceBlock=sps_lib/Power Grid Elements/Distributed Parameters Line
  TEST1-PNS 235 km : spsDistributedParametersLineLib/Distributed Parameters Line  Phases=3  Length=235  Frequency=60  Resistance=[0.01273 0.3864]/6  Inductance="[0.9337e-3  4.1264e-3]/6"  Capacitance=[12.74e-9 7.751e-9]*6  x1=[-0.00138 -1.73849812036604e-12 -0.314411797067839 1.83038122760652;-0.00132 -1.74658907605976e-12 -0.355531650273569 1.8227836062879;-0.00126 -1.75378644450891e-12 -0.39646960691755 1.81425341519512;-0.0012 -1.7600865434068e-12 -0.437204722384716 1.80479501853159;-0.00114 -1.76548614950643e-12 -0.477716155837295 1.7944132553878;-0.00108 -1.76998250026953e-12 -0.517983180877368 1.78311343726561;-0.00102 -1.77357329527998e-12 -0.557985196150876 1.77090134536076;-0.00096 -1.7762566974207e-12 -0.597701735887652 1.75778322760513;-0.0009 -1.77803133381356e-12 -0.63711248037209 1.74376579547016;-0.00084 -1.77889629652181e-12 -0.676197266339084 1.72885622053314;-0.00078 -1.77885114301453e-12 -0.71493609728993 1.71306213080811;-0.00072 -1.7778958963931e-12 -0.753309153722903 1.6963916068432;-0.00066 -1.77603104537933e-12 -0.791296803273277 1.67885317758653;-0.0006 -1.77325754406547e-12 -0.828879610757614 1.66045581602255;-0.00054 -1.76957681142603e-12 -0.866038348117153 1.64120893458141;-0.00048 -1.76499073059184e-12 -0.902754004255247 1.62112238032328;-0.00042 -1.75950164788661e-12 -0.939007794763787 1.60020642990048;-0.00036 -1.75311237162646e-12 -0.974781171533657 1.57847178429972;-0.0003 -1.7458261706832e-12 -1.01005583224429 1.55592956336732;-0.00024 -1.73764677281185e-12 -1.04481372972745 1.53259130012002;-0.00018 -1.72857836274352e-12 -1.07903708120055 1.50846893484455;-0.00012 -1.71862558004435e-12 -1.1127083773646 1.48357480898871;-6e-05 -1.70779351674188e-12 -1.1458103913623 1.45792165884728]  x2=[-0.00138 3.68525736767454e-13 1.78181025544666 -5.47262183729712;-0.00132 3.67945428890442e-13 1.9045190703255 -5.43074679883814;-0.00126 3.6717687333316e-13 2.02625349805649 -5.38609328996821;-0.0012 3.66220463302832e-13 2.14695125705702 -5.33868415624757;-0.00114 3.65076688116503e-13 2.26655059612334 -5.28854365306506;-0.00108 3.63746132950691e-13 2.38499032602364 -5.23569743322858;-0.00102 3.62229478542006e-13 2.5022098508036 -5.1801725338407;-0.00096 3.60527500838868e-13 2.61814919878836 -5.12199736246593;-0.0009 3.58641070604518e-13 2.73274905326519 -5.06120168259688;-0.00084 3.56571152971522e-13 2.84595078283097 -4.99781659842677;-0.00078 3.54318806947988e-13 2.95769647138913 -4.93187453893587;-0.00072 3.51885184875761e-13 3.06792894778058 -4.86340924130028;-0.00066 3.49271531840861e-13 3.17659181503354 -4.79245573363138;-0.0006 3.46479185036475e-13 3.28362947921725 -4.71905031705475;-0.00054 3.43509573078826e-13 3.38898717788491 -4.64323054713789;-0.00048 3.40364215276262e-13 3.49261100809107 -4.56503521467608;-0.00042 3.37044720851955e-13 3.59444795396947 -4.48450432584628;-0.00036 3.3355278812059e-13 3.69444591385685 -4.40167908173928;-0.0003 3.29890203619475e-13 3.79255372694919 -4.31660185728037;-0.00024 3.26058841194519e-13 3.88872119947648 -4.22931617954966;-0.00018 3.22060661041533e-13 3.98289913038283 -4.1398667055127;-0.00012 3.17897708703362e-13 4.07503933649855 -4.04829919917326;-6e-05 3.13572114023343e-13 4.16509467719165 -3.95466050815956]  x3=[-0.00138 -1.01291248713011e-14 -0.527069956693164 -0.131666817190006;-0.00132 -9.51541533487076e-15 -0.523968959751768 -0.143612734919043;-0.00126 -8.89683753613038e-15 -0.52059989060873 -0.155485177719237;-0.0012 -8.27370795091187e-15 -0.516964472942077 -0.167278071429474;-0.00114 -7.64634538382513e-15 -0.513064566698662 -0.178985382587425;-0.00108 -7.0150708051518e-15 -0.50890216714258 -0.190601121516374;-0.00102 -6.38020718663096e-15 -0.504479403834357 -0.202119345389652;-0.00096 -5.74207933622076e-15 -0.499798539541425 -0.213534161271092;-0.0009 -5.10101373192072e-15 -0.494861969080449 -0.224839729129968;-0.00084 -4.45733835473953e-15 -0.489672218092093 -0.236030264828861;-0.00078 -3.81138252089392e-15 -0.484231941748859 -0.24710004308293;-0.00072 -3.16347671332437e-15 -0.478543923396649 -0.258043400389073;-0.00066 -2.51395241261395e-15 -0.472611073130754 -0.268854737923484;-0.0006 -1.86314192739673e-15 -0.466436426306996 -0.279528524406109;-0.00054 -1.21137822434256e-15 -0.460023141988786 -0.290059298930554;-0.00048 -5.58994757805119e-16 -0.453374501330884 -0.300441673757987;-0.00042 9.36747007794521e-17 -0.446493905900704 -0.310670337073601;-0.00036 7.46296233656195e-16 -0.439384875938006 -0.320740055704241;-0.0003 1.39853594758983e-15 -0.432051048553879 -0.330645677795788;-0.00024 2.05006014469071e-15 -0.424496175869926 -0.340382135448944;-0.00018 2.7005354931408e-15 -0.416724123098611 -0.349944447312066;-0.00012 3.34962919773245e-15 -0.408738866565743 -0.359327721129714;-6e-05 3.9970091701325e-15 -0.400544491676113 -0.368527156245619]  x4=[-0.00138 6.15082186092157e-16 0.547022847111482 0.0466107611971553;-0.00132 -1.24909215055942e-16 0.545830869396191 0.0590317620219681;-0.00126 -8.64836710341563e-16 0.544359634522321 0.0714225611065491;-0.0012 -1.60432173918583e-15 0.542609895200821 0.0837768190891307;-0.00114 -2.34298596738386e-15 0.540582546630658 0.0960882153030487;-0.00108 -3.08045148066759e-15 0.538278626040821 0.108350451010512;-0.00102 -3.8163409780536e-15 0.535699312159657 0.120557252625151;-0.00096 -4.55027796487737e-15 0.532845924611806 0.132702374921706;-0.0009 -5.28188694541484e-15 0.529719923243064 0.144779604231193;-0.00084 -6.01079361499298e-15 0.526322907373492 0.156782761619936;-0.00078 -6.736625051491e-15 0.522656614979178 0.168705706050822;-0.00072 -7.45900990613416e-15 0.518722921803057 0.180542337525169;-0.00066 -8.17757859348267e-15 0.514523840395244 0.192286600203599;-0.0006 -8.89196348051849e-15 0.510061519083377 0.203932485504317;-0.00054 -9.60179907473309e-15 0.505338240873494 0.215474035177212;-0.00048 -1.03067222111202e-14 0.500356422282003 0.226905344352209;-0.00042 -1.10063722379778e-14 0.495118612099349 0.238220564560306;-0.00036 -1.1700391201424e-14 0.489627490086005 0.249413906725763;-0.0003 -1.23884240285332e-14 0.483885865601457 0.260479644127901;-0.00024 -1.30701187089977e-14 0.477896676166885 0.271412115330993;-0.00018 -1.37451264752226e-14 0.47166298596227 0.282205727080762;-0.00012 -1.44131019807621e-14 0.465187984258707 0.292854957165994;-6e-05 -1.50737034770047e-14 0.458474983786712 0.303354357243803]  x5=0.00132902268243999  V1=[4.457e-19 3.159e-07 3.159e-07;377 377 377;1.774 1.251 -0.3202]  V2=[2.934e-17 4.144e-06 4.144e-06;377 377 377;-1.608 -1.933 2.78]  I1=[7.734e-20 5.426e-08 5.426e-08;377 377 377;-2.952 2.797 1.226]  I2=[6.83e-20 5.366e-08 5.366e-08;377 377 377;-0.313 -0.6082 -2.179]  nHarmo=1  Measurements=None  Decoupling=off  VsMag0=0  VrMag0=0  VsAngle0=0  VrAngle0=0  IsMag0=0  IrMag0=0  IsAngle0=0  IrAngle0=0
      settings: LibrarySourceBlock=sps_lib/Power Grid Elements/Distributed Parameters Line
  TEST2 : spsThreePhaseVIMeasurementLib/Three-Phase V-I Measurement  VoltageMeasurement=no  SetLabelV=off  LabelV=Vabc  Vpu=off  VpuLL=off  CurrentMeasurement=no  SetLabelI=off  LabelI=Iabc  Ipu=off  Pbase=100e6  Vbase=500e3  OutputType=Complex  PhasorSimulation=off  PSBequivalent=0
  CON-a : PMIOPort  Side=Left
  CON-b : PMIOPort  Port=2  Side=Left
  CON-c : PMIOPort  Port=3  Side=Left
  SAT-a : PMIOPort  Port=4  Side=Left
  SAT-b : PMIOPort  Port=5  Side=Left
  SAT-c : PMIOPort  Port=6  Side=Left
  wires:
  Regulators 1/2(Vf) -> MPP1_3700MVA 17KV/2
  Regulators 1/1(Pm) -> MPP1_3700MVA 17KV/1
  Regulators 4/1(Pm) -> MPP4_3800MVA 17KV/1
  Regulators 4/2(Vf) -> MPP4_3800MVA 17KV/2
  MPP1_3700MVA 17KV/1 -> Regulators 1/1(m)
  Regulators 3/1(Pm) -> MPP3_800MVA 17KV/1
  Regulators 2/1(Pm) -> MPP2_500MVA 17KV/1
  MPP4_3800MVA 17KV/1 -> Regulators 4/1(m)
  MPP3_800MVA 17KV/1 -> Regulators 3/1(m)
  Regulators 3/2(Vf) -> MPP3_800MVA 17KV/2
  Regulators 2/2(Vf) -> MPP2_500MVA 17KV/2
  MPP2_500MVA 17KV/1 -> Regulators 2/1(m)
  Regulators 5/1(Pm) -> MPP5_4200MVA 17KV/1
  Regulators 5/2(Vf) -> MPP5_4200MVA 17KV/2
  MPP5_4200MVA 17KV/1 -> Regulators 5/1(m)
  Regulators 6/1(Pm) -> MPP6_490MVA 17KV/1
  Regulators 6/2(Vf) -> MPP6_490MVA 17KV/2
  MPP6_490MVA 17KV/1 -> Regulators 6/1(m)
  connections:
  CLP-CSG 103 km/LConn3 -- Cs CSGN/LConn3
  CLP-TEST2 288 km/RConn1 -- Cs CLPS/LConn1 -- Cs AND/RConn1
  CLP 1/LConn3 -- 4200 MVA 17KV :650KV Transformer/RConn3 -- Cs CLPN/RConn3 -- Cs CLPS/RConn3
  "500 MVA 17KV :650KV Transformer "/LConn3 -- 1980 MVar/LConn3 -- TEST1-MPP2 187 km/LConn1
  CLP-CSG 103 km/RConn1 -- 990 MVar3/LConn1 -- CLP 1/RConn1 -- Load Flow Bus7/LConn1
  MPP3-TEST2 111 km/RConn2 -- 660 MVar4/LConn2 -- MPP4-TEST2 96 km/RConn2 -- TEST2/LConn2
  MPP2_500MVA 17KV/RConn2 -- 25 MW/LConn2 -- "500 MVA 17KV :650KV Transformer "/RConn2
  TEST1-PNS 235 km/LConn2 -- TEST 1/LConn2 -- TEST1-MPP2 187 km/RConn2
  "3700 MVA 17KV :650KV Transformer "/LConn3 -- MPP1_3700MVA 17KV/RConn3 -- 185 MW/LConn3
  "500 MVA 17KV :650KV Transformer "/RConn3 -- 25 MW/LConn3 -- MPP2_500MVA 17KV/RConn3
  40 MW/LConn1 -- MPP3_800MVA 17KV/RConn1 -- 800 MVA 17KV :650KV Transformer/RConn1 -- Load Flow Bus4/LConn1
  MPP4_3800MVA 17KV/RConn1 -- 190 MW/LConn1 -- Load Flow Bus6/LConn1 -- 3800 MVA 17KV :650KV Transformer/RConn1
  "500 MVA 17KV :650KV Transformer "/LConn1 -- 1980 MVar/LConn1 -- TEST1-MPP2 187 km/LConn3
  CLP 1/RConn3 -- 990 MVar3/LConn3 -- CLP-CSG 103 km/RConn3
  Cs CSGN/LConn2 -- CLP-CSG 103 km/LConn2
  MPP4_3800MVA 17KV/RConn3 -- 190 MW/LConn3 -- 3800 MVA 17KV :650KV Transformer/RConn3
  "3700 MVA 17KV :650KV Transformer "/LConn1 -- Load Flow Bus/LConn1 -- 185 MW/LConn1 -- MPP1_3700MVA 17KV/RConn1
  CLP 1/LConn1 -- 4200 MVA 17KV :650KV Transformer/RConn1 -- Cs CLPN/RConn1 -- Cs CLPS/RConn1
  CLP 1/LConn2 -- 4200 MVA 17KV :650KV Transformer/RConn2 -- Cs CLPN/RConn2 -- Cs CLPS/RConn2
  3800 MVA 17KV :650KV Transformer/LConn2 -- MPP4-TEST2 96 km/LConn2
  "3700 MVA 17KV :650KV Transformer "/RConn1 -- MPP1-CLP 310 km/LConn1 -- Cs MPP1D/RConn1 -- 1320 MVar/LConn1 -- Load Flow Bus2/LConn1
  3800 MVA 17KV :650KV Transformer/LConn1 -- Load Flow Bus3/LConn1 -- MPP4-TEST2 96 km/LConn1
  "3700 MVA 17KV :650KV Transformer "/LConn2 -- 185 MW/LConn2 -- MPP1_3700MVA 17KV/RConn2
  MPP3-TEST2 111 km/RConn3 -- 660 MVar4/LConn1 -- MPP4-TEST2 96 km/RConn3 -- TEST2/LConn3
  TEST1-MPP2 187 km/RConn1 -- TEST 1/LConn3 -- TEST1-PNS 235 km/LConn3
  TEST2/RConn3 -- CLP-TEST2 288 km/LConn3
  MPP3-TEST2 111 km/RConn1 -- 660 MVar4/LConn3 -- MPP4-TEST2 96 km/RConn1 -- TEST2/LConn1
  Cs CLPS/LConn2 -- Cs AND/RConn2 -- CLP-TEST2 288 km/RConn2
  CLP-TEST2 288 km/RConn3 -- Cs CLPS/LConn3 -- Cs AND/RConn3
  800 MVA 17KV :650KV Transformer/LConn2 -- MPP3-TEST2 111 km/LConn2
  CSG 1/LConn3 -- Cs CSGN/RConn3
  MPP4_3800MVA 17KV/RConn2 -- 190 MW/LConn2 -- 3800 MVA 17KV :650KV Transformer/RConn2
  800 MVA 17KV :650KV Transformer/RConn2 -- 40 MW/LConn2 -- MPP3_800MVA 17KV/RConn2
  800 MVA 17KV :650KV Transformer/LConn1 -- MPP3-TEST2 111 km/LConn1
  MPP1-CLP 310 km/RConn1 -- Cs CLPN/LConn1
  MPP1-CLP 310 km/RConn3 -- Cs CLPN/LConn3
  TEST1-MPP2 187 km/LConn2 -- 1980 MVar/LConn2 -- "500 MVA 17KV :650KV Transformer "/LConn2
  TEST2/RConn1 -- Load Flow Bus5/LConn1 -- CLP-TEST2 288 km/LConn1
  MPP2_500MVA 17KV/RConn1 -- Load Flow Bus1/LConn1 -- 25 MW/LConn1 -- "500 MVA 17KV :650KV Transformer "/RConn1
  800 MVA 17KV :650KV Transformer/LConn3 -- MPP3-TEST2 111 km/LConn3
  MPP1-CLP 310 km/RConn2 -- Cs CLPN/LConn2
  CLP-CSG 103 km/RConn2 -- 990 MVar3/LConn2 -- CLP 1/RConn2
  CSG 1/LConn2 -- Cs CSGN/RConn2
  MPP3_800MVA 17KV/RConn3 -- 40 MW/LConn3 -- 800 MVA 17KV :650KV Transformer/RConn3
  CSG 1/LConn1 -- Cs CSGN/RConn1
  TEST2/RConn2 -- CLP-TEST2 288 km/LConn2
  3800 MVA 17KV :650KV Transformer/LConn3 -- MPP4-TEST2 96 km/LConn3
  Cs CSGN/LConn1 -- CLP-CSG 103 km/LConn1
  MPP5_4200MVA 17KV/RConn1 -- 210 MW/LConn1 -- 4200 MVA 17KV :650KV Transformer/LConn1 -- Load Flow Bus10/LConn1
  MPP5_4200MVA 17KV/RConn2 -- 210 MW/LConn2 -- 4200 MVA 17KV :650KV Transformer/LConn2
  MPP5_4200MVA 17KV/RConn3 -- 210 MW/LConn3 -- 4200 MVA 17KV :650KV Transformer/LConn3
  MPP6_490MVA 17KV/RConn1 -- 25 MW1/LConn1 -- 490 MVA 17KV :650KV Transformer/LConn1 -- Load Flow Bus12/LConn1
  MPP6_490MVA 17KV/RConn2 -- 25 MW1/LConn2 -- 490 MVA 17KV :650KV Transformer/LConn2
  MPP6_490MVA 17KV/RConn3 -- 25 MW1/LConn3 -- 490 MVA 17KV :650KV Transformer/LConn3
  Cs PNSM/LConn3 -- PNS3/RConn3
  Cs PNSM/LConn1 -- PNS3/RConn1
  Cs PNSM/LConn2 -- PNS3/RConn2
  Cs PNSN/RConn2 -- PNS3/LConn2
  PNS3/LConn3 -- Cs PNSN/RConn3
  Cs PNSN/RConn1 -- PNS3/LConn1 -- Load Flow Bus8/LConn1
  490 MVA 17KV :650KV Transformer/RConn1 -- 2310 MVar/LConn1 -- MPP6-CSG 186 km/LConn1
  490 MVA 17KV :650KV Transformer/RConn2 -- 2310 MVar/LConn2 -- MPP6-CSG 186 km/LConn2
  MPP6-CSG 186 km/RConn1 -- CSG 1/RConn1
  MPP6-CSG 186 km/RConn2 -- CSG 1/RConn2
  MPP6-CSG 186 km/RConn3 -- CSG 1/RConn3
  490 MVA 17KV :650KV Transformer/RConn3 -- 2310 MVar/LConn3 -- MPP6-CSG 186 km/LConn3
  SAT-a/RConn1 -- 660 MVar/LConn1 -- Cs SATS/RConn1
  SAT-b/RConn1 -- 660 MVar/LConn2 -- Cs SATS/RConn2
  SAT-c/RConn1 -- 660 MVar/LConn3 -- Cs SATS/RConn3
  Cs SATS/LConn3 -- " SAT-AND 129 km"/LConn3
  " SAT-AND 129 km"/LConn1 -- Cs SATS/LConn1
  Cs SATS/LConn2 -- " SAT-AND 129 km"/LConn2
  Cs PNSM/RConn1 -- TEST1-PNS 235 km/RConn1
  TEST1-PNS 235 km/RConn2 -- Cs PNSM/RConn2
  Cs PNSM/RConn3 -- TEST1-PNS 235 km/RConn3
  PNS-CON 260 km/LConn1 -- 990 MVar/LConn1 -- Cs PNSN/LConn1
  PNS-CON 260 km/LConn2 -- 990 MVar/LConn2 -- Cs PNSN/LConn2
  PNS-CON 260 km/LConn3 -- 990 MVar/LConn3 -- Cs PNSN/LConn3
  CON-a/RConn1 -- PNS-CON 260 km/RConn1
  CON-b/RConn1 -- PNS-CON 260 km/RConn2
  CON-c/RConn1 -- PNS-CON 260 km/RConn3
  AND1/RConn3 -- " SAT-AND 129 km"/RConn3
  AND1/RConn2 -- " SAT-AND 129 km"/RConn2
  AND1/RConn1 -- " SAT-AND 129 km"/RConn1
  Cs AND/LConn1 -- AND1/LConn1
  Cs AND/LConn3 -- Load Flow Bus11/LConn1 -- AND1/LConn3
  Cs AND/LConn2 -- AND1/LConn2
  TEST1-PNS 235 km/LConn1 -- TEST 1/LConn1 -- TEST1-MPP2 187 km/RConn3
  "3700 MVA 17KV :650KV Transformer "/RConn2 -- Cs MPP1D/RConn2 -- 1320 MVar/LConn2 -- MPP1-CLP 310 km/LConn2
  MPP1-CLP 310 km/LConn3 -- Cs MPP1D/RConn3 -- 1320 MVar/LConn3 -- "3700 MVA 17KV :650KV Transformer "/RConn3
  TEST 1/RConn1 -- Cs MPP1D/LConn1
  TEST 1/RConn2 -- Cs MPP1D/LConn2
  TEST 1/RConn3 -- Cs MPP1D/LConn3
